simulink model "Gripper2"  (R2013b)
settings: Solver=ode45  StartTime=0.0  StopTime=6  RelTol=1e-3
undefined symbols (not defined in the file): base, driveshaft, grip, GripperForSimulink, link1, link2, link3, link4, Part8, pin1, pin15mm, pin50mm, RootGround, RootPart
libraries: mblibv1 x65, fl_lib x10, nesl_utility x5, elec_lib x1, simulink x1
(part 2 of 2)

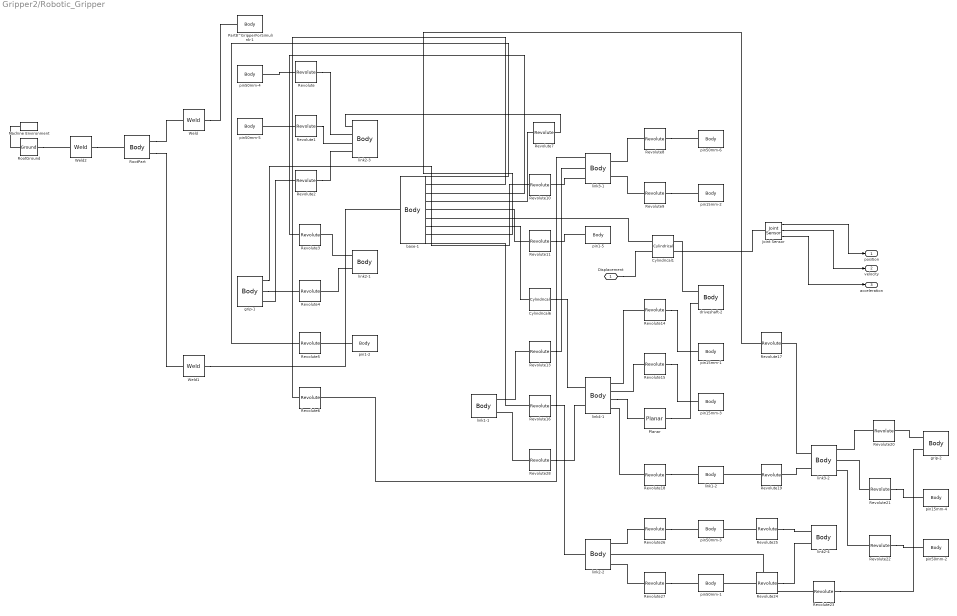
== system Gripper2/Robotic_Gripper ==
  Cylindrical1 : mblibv1/Joints/Cylindrical  LConnTagsString=__newl0|SA1  RConnTagsString=__newr0|SA1  UpdateFromCAD=on  NumSAPorts=2  CutJoint=off  MarkAsCut=off  Primitives=prismatic  PrimitiveProps=P1$World$[1 0 0]$prismatic#R1$World$[1 0 0]$revolute  DialogClass=JointBlock  P1Axis=[1 0 0]  R1Axis=[1 0 0]
  Cylindrical6 : mblibv1/Joints/Cylindrical  LConnTagsString=__newl0  RConnTagsString=__newr0  UpdateFromCAD=on  PMImportedID=base-1:-:link4-1  NumSAPorts=0  CutJoint=off  MarkAsCut=off  Primitives=prismatic  PrimitiveProps=P1$World$[1 0 0]$prismatic#R1$World$[1 0 0]$revolute  DialogClass=JointBlock  P1Axis=[1 0 0]  R1Axis=[1 0 0]
  Joint Sensor : mblibv1/Sensors &  Actuators/Joint Sensor  UpdateFromCAD=off  PhysicalDomain=Mechanical  PortType=blob  Muxed=off  Pose=off  Angle=on  AngleUnits=deg  ArcVelocity=off  ArcVelocityUnits=deg/s  ArcAcceleration=off  ArcAccelerationUnits=deg/s^2  CoordPosition=on  CoordPositionUnits=m  Velocity=on  VelocityUnits=m/s  Acceleration=on  AccelerationUnits=m/s^2  Quaternion=on  QuaternionDT=off  QuaternionDDT=off  QuaternionUnits=off  OutputVector=[1]  ActiveIO=on  Width=3  DialogClass=MechanicalSensorBlock  Primitive=P1  Force=off  ForceUnits=N  Torque=off  TorqueUnits=N*m  ReferenceFrame=Absolute (World)  ReactionSensedSide=Base  ReactionReferenceFrame=Absolute (World)  ReactionForce=off  ReactionForceUnits=N  ReactionMoment=off  ReactionMomentUnits=N*m
  Machine Environment : mblibv1/Bodies/Machine Environment  PortType=env  PhysicalDomain=Mechanical  DialogTemplateClass=MECH.MachineEnvironment  SyncWhenCopied=off  Gravity=[0 0 0]  GravityUnits=m/s^2  GravityAsSignal=off  Dimensionality=Auto-detect  AnalysisType=Forward dynamics  LinearAssemblyTolerance=1e-3  LinearAssemblyToleranceUnits=m  AngularAssemblyTolerance=1e-3  AngularAssemblyToleranceUnits=rad  ConstraintSolverType=Stabilizing  ConstraintRelTolerance=1e-4  ConstraintAbsTolerance=1e-4  UseRobustSingularityHandling=off  RedundancyAnalysisToleranceType=Automatically select tolerance  RedundancyAnalysisTolerance=1e-14  StatePerturbationType=Fixed  PerturbationSize=1e-5  VisualizeMachine=on  BodyVisualizationType=Use model default body geometries  BodyColorSelMode=Use model default  DefaultBodyColor=[1 0 0]
  Part8^GripperForSimulink-1 : mblibv1/Bodies/Body  LConnTagsString=CS2  UpdateFromCAD=on  PMImportedID=Part8^GripperForSimulink-1  DialogClass=MechanicalBodyBlock  Mass=0  MassUnits=kg  InertiaUnits=kg*m^2  Inertia=[0,0,0;0,0,0;0,0,0]  Shape=Cylinder  ShapeDims=[1 1]  ShapeUnits=m  ShapeUse=false  Density=1  DensityUnits=kg/m^3  DensityUse=false  GraphicsMode=GFXFILE  GraphicsFileName=GripperForSimulink - Part8^GripperForSimulink-1.STL  BodyColorSelMode=COLORPALETTE  BodyColor=[0.792157;0.819608;0.933333]  AttachedToCS=CS1  CG=Right$CG$[0 0 0]$WORLD$WORLD$m$[1 0 0;0 1 0;0 0 1]$3x3 Transform$rad$WORLD$false$Part8^GripperForSimulink-1::CG(AUTOGEN)  WorkingFrames=Right$CS1$[0 0 0]$WORLD$WORLD$m$[1 0 0;0 1 0;0 0 1]$3x3 Transform$rad$WORLD$false$Part8^GripperForSimulink-1::CS1(AUTOGEN)#Left$CS2$[0 0 0]$WORLD$WORLD$m$[1 0 0;0 1 0;0 0 1]$3x3 Transform$rad$WORLD$true$GripperForSimulink/RootPart:-:Part8^GripperForSimulink-1::Part8^GripperForSimulink-1(AUTOGEN)  CGPos=[0 0 0]  CGRot=[1 0 0;0 1 0;0 0 1]  CS0Pos=[]  CS0Rot=[]  CS1Pos=[0 0 0]  CS1Rot=[1 0 0;0 1 0;0 0 1]  CS2Pos=[0 0 0]  CS2Rot=[1 0 0;0 1 0;0 0 1]  CS3Pos=[]  CS3Rot=[]  CS4Pos=[]  CS4Rot=[]  CS5Pos=[]  CS5Rot=[]  CS6Pos=[]  CS6Rot=[]  CS7Pos=[]  CS7Rot=[]  CS8Pos=[]  CS8Rot=[]  CS9Pos=[]  CS9Rot=[]  CS10Pos=[]  CS10Rot=[]  CS11Pos=[]  CS11Rot=[]  CS12Pos=[]  CS12Rot=[]  CS13Pos=[]  CS13Rot=[]  CS14Pos=[]  CS14Rot=[]  CS15Pos=[]  CS15Rot=[]  CS16Pos=[]  CS16Rot=[]  CS17Pos=[]  CS17Rot=[]  CS18Pos=[]  CS18Rot=[]  CS19Pos=[]  CS19Rot=[]  CS20Pos=[]  CS20Rot=[]
  Planar : mblibv1/Joints/Planar  LConnTagsString=__newl0  RConnTagsString=__newr0  UpdateFromCAD=on  PMImportedID=driveshaft-2:-:link4-1  NumSAPorts=0  CutJoint=off  MarkAsCut=off  Primitives=prismatic_prismatic  PrimitiveProps=P1$World$[0,1,0]$prismatic#P2$World$[0,0,1]$prismatic#R1$World$[1,0,0]$revolute  DialogClass=JointBlock  P1Axis=[0,1,0]  P2Axis=[0,0,1]  R1Axis=[1,0,0]
  Revolute{,1..11,13..28} (28 alike) : mblibv1/Joints/Revolute  LConnTagsString=__newl0  RConnTagsString=__newr0  UpdateFromCAD=off  NumSAPorts=0  CutJoint=off  MarkAsCut=off  Primitives=prismatic  PrimitiveProps=R1$WORLD$[0 0 1]$revolute  DialogClass=JointBlock  R1Axis=[0 0 1]
  RootGround : mblibv1/Bodies/Ground  UpdateFromCAD=on  PMImportedID=RootGround  LeftPortType=env  RightPortType=workingframe  PhysicalDomain=Mechanical  DialogClass=GroundBlock  CoordPosition=[0.0300865,-0.00078351,0.0233471]  CoordPositionUnits=m  StateVectorMgrId=4  MachineId=[5 0]  ShowEnvPort=on  ParameterChecksum=[2079004459, 1115045925, 2663181990, 1030677230]  TopologyChecksum=[1966038930, 1606209126, 1995956594, 3418706587]
  RootPart : mblibv1/Bodies/Body  LConnTagsString=CS4  RConnTagsString=CS2|CS3  UpdateFromCAD=on  PMImportedID=GripperForSimulink/RootPart  DialogClass=MechanicalBodyBlock  Mass=0  MassUnits=kg  InertiaUnits=kg*m^2  Inertia=[0,0,0;0,0,0;0,0,0]  Shape=Cylinder  ShapeDims=[1 1]  ShapeUnits=m  ShapeUse=false  Density=1  DensityUnits=kg/m^3  DensityUse=false  GraphicsMode=MACHINE_DEFAULT  BodyColorSelMode=MACHINE_DEFAULT  BodyColor=[1;0;0]  AttachedToCS=CS1  CG=Right$CG$[0.0300865 -0.00078351 0.0233471]$WORLD$WORLD$m$[1 0 0;0 1 0;0 0 1]$3x3 Transform$rad$WORLD$false$GripperForSimulink/RootPart::CG(AUTOGEN)  WorkingFrames=Right$CS1$[0 0 0]$WORLD$WORLD$m$[1 0 0;0 1 0;0 0 1]$3x3 Transform$rad$WORLD$false$GripperForSimulink/RootPart::CS1(AUTOGEN)#Right$CS2$[0 0 0]$WORLD$WORLD$m$[1 0 0;0 1 0;0 0 1]$3x3 Transform$rad$WORLD$true$GripperForSimulink/RootPart:-:Part8^GripperForSimulink-1::GripperForSimulink/RootPart(AUTOGEN)#Right$CS3$[-0.043944 -0.000782836 0.0233426]$WORLD$WORLD$m$[1 0 0;0 1 0;0 0 1]$3x3 Transform$rad$WORLD$true$GripperForSimulink/RootPart:-:base-1::GripperForSimulink/RootPart(AUTOGEN)#Left$CS4$[0.0300865 -0.00078351 0.0233471]$WORLD$WORLD$m$[1 0 0;0 1 0;0 0 1]$3x3 Transform$rad$WORLD$true$GripperForSimulink/RootPart:-:RootGround::GripperForSimulink/RootPart(AUTOGEN)  CGPos=[0.0300865 -0.00078351 0.0233471]  CGRot=[1 0 0;0 1 0;0 0 1]  CS0Pos=[]  CS0Rot=[]  CS1Pos=[0 0 0]  CS1Rot=[1 0 0;0 1 0;0 0 1]  CS2Pos=[0 0 0]  CS2Rot=[1 0 0;0 1 0;0 0 1]  CS3Pos=[-0.043944 -0.000782836 0.0233426]  CS3Rot=[1 0 0;0 1 0;0 0 1]  CS4Pos=[0.0300865 -0.00078351 0.0233471]  CS4Rot=[1 0 0;0 1 0;0 0 1]  CS5Pos=[]  CS5Rot=[]  CS6Pos=[]  CS6Rot=[]  CS7Pos=[]  CS7Rot=[]  CS8Pos=[]  CS8Rot=[]  CS9Pos=[]  CS9Rot=[]  CS10Pos=[]  CS10Rot=[]  CS11Pos=[]  CS11Rot=[]  CS12Pos=[]  CS12Rot=[]  CS13Pos=[]  CS13Rot=[]  CS14Pos=[]  CS14Rot=[]  CS15Pos=[]  CS15Rot=[]  CS16Pos=[]  CS16Rot=[]  CS17Pos=[]  CS17Rot=[]  CS18Pos=[]  CS18Rot=[]  CS19Pos=[]  CS19Rot=[]  CS20Pos=[]  CS20Rot=[]
  Weld : mblibv1/Joints/Weld  LConnTagsString=__newl0  RConnTagsString=__newr0  UpdateFromCAD=on  PMImportedID=GripperForSimulink/RootPart:-:Part8^GripperForSimulink-1  NumSAPorts=0  CutJoint=off  MarkAsCut=off  Primitives=weld  PrimitiveProps=W$WORLD$[0.57735,0.57735,0.57735]$weld  DialogClass=JointBlock  WAxis=[0.57735,0.57735,0.57735]
  Weld1 : mblibv1/Joints/Weld  LConnTagsString=__newl0  RConnTagsString=__newr0  UpdateFromCAD=on  PMImportedID=GripperForSimulink/RootPart:-:base-1  NumSAPorts=0  CutJoint=off  MarkAsCut=off  Primitives=weld  PrimitiveProps=W$WORLD$[0.57735,0.57735,0.57735]$weld  DialogClass=JointBlock  WAxis=[0.57735,0.57735,0.57735]
  Weld2 : mblibv1/Joints/Weld  LConnTagsString=__newl0  RConnTagsString=__newr0  UpdateFromCAD=on  PMImportedID=GripperForSimulink/RootPart:-:RootGround  NumSAPorts=0  CutJoint=off  MarkAsCut=off  Primitives=weld  PrimitiveProps=W$WORLD$[0.57735,0.57735,0.57735]$weld  DialogClass=JointBlock  WAxis=[0.57735,0.57735,0.57735]
  base-1 : mblibv1/Bodies/Body  LConnTagsString=CS2  RConnTagsString=CS3|CS4|CS5|CS6|CS7|CS8|CS9|CS10|CS11  UpdateFromCAD=on  PMImportedID=base-1  DialogClass=MechanicalBodyBlock  Mass=0.147606  MassUnits=kg  InertiaUnits=kg*m^2  Inertia=[0.000194575,0,0;0,0.000219515,0;0,0,0.000354174]  Shape=Cylinder  ShapeDims=[1 1]  ShapeUnits=m  ShapeUse=false  Density=1  DensityUnits=kg/m^3  DensityUse=false  GraphicsMode=GFXFILE  GraphicsFileName=GripperForSimulink - base-1.STL  BodyColorSelMode=COLORPALETTE  BodyColor=[0.792157;0.819608;0.933333]  AttachedToCS=CS1  CG=Right$CG$[-0.043944 -0.000782836 0.0233426]$WORLD$WORLD$m$[1 0 0;0 1 0;0 0 1]$3x3 Transform$rad$WORLD$false$base-1::CG(AUTOGEN)  WorkingFrames=Right$CS1$[6.48367e-05 0.0413573 0.00359264]$WORLD$WORLD$m$[1 0 0;0 1 0;0 0 1]$3x3 Transform$rad$WORLD$false$base-1::CS1(AUTOGEN)#Left$CS2$[-0.043944 -0.000782836 0.0233426]$WORLD$WORLD$m$[1 0 0;0 1 0;0 0 1]$3x3 Transform$rad$WORLD$true$GripperForSimulink/RootPart:-:base-1::base-1(AUTOGEN)#Right$CS3$[-0.00973859 0.0614627 0.0108426]$WORLD$WORLD$m$[1 0 0;0 1 0;0 0 1]$3x3 Transform$rad$WORLD$true$base-1:-:pin1-2::base-1(AUTOGEN)#Right$CS4$[-0.00973859 0.0614627 0.0358426]$WORLD$WORLD$m$[1 0 0;0 1 0;0 0 1]$3x3 Transform$rad$WORLD$true$base-1:-:link3-1::base-1(AUTOGEN)#Right$CS5$[0.00656063 0.0362648 0.0358426]$WORLD$WORLD$m$[1 0 0;0 1 0;0 0 1]$3x3 Transform$rad$WORLD$true$base-1:-:link2-1::base-1(AUTOGEN)#Right$CS6$[0.00656063 0.0362648 0.0108426]$WORLD$WORLD$m$[1 0 0;0 1 0;0 0 1]$3x3 Transform$rad$WORLD$true$base-1:-:link2-3::base-1(AUTOGEN)#Right$CS7$[-0.00973859 -0.0630284 0.0358426]$WORLD$WORLD$m$[1 0 0;0 1 0;0 0 1]$3x3 Transform$rad$WORLD$true$base-1:-:pin1-5::base-1(AUTOGEN)#Right$CS8$[0.0165606 -0.000782836 0.0233426]$WORLD$WORLD$m$[1 0 0;0 1 0;0 0 1]$3x3 Transform$rad$WORLD$true$base-1:-:driveshaft-2::base-1(AUTOGEN)#Right$CS9$[0.0165606 -0.000782836 0.0233426]$WORLD$WORLD$m$[1 0 0;0 1 0;0 0 1]$3x3 Transform$rad$WORLD$true$base-1:-:link4-1::base-1(AUTOGEN)#Right$CS10$[-0.00973859 -0.0630284 0.0358426]$WORLD$WORLD$m$[1 0 0;0 1 0;0 0 1]$3x3 Transform$rad$WORLD$true$base-1:-:link3-2::base-1(AUTOGEN)#Right$CS11$[0.00656063 -0.0378305 0.0108426]$WORLD$WORLD$m$[1 0 0;0 1 0;0 0 1]$3x3 Transform$rad$WORLD$true$base-1:-:link2-2::base-1(AUTOGEN)  CGPos=[-0.043944 -0.000782836 0.0233426]  CGRot=[1 0 0;0 1 0;0 0 1]  CS0Pos=[]  CS0Rot=[]  CS1Pos=[6.48367e-05 0.0413573 0.00359264]  CS1Rot=[1 0 0;0 1 0;0 0 1]  CS2Pos=[-0.043944 -0.000782836 0.0233426]  CS2Rot=[1 0 0;0 1 0;0 0 1]  CS3Pos=[-0.00973859 0.0614627 0.0108426]  CS3Rot=[1 0 0;0 1 0;0 0 1]  CS4Pos=[-0.00973859 0.0614627 0.0358426]  CS4Rot=[1 0 0;0 1 0;0 0 1]  CS5Pos=[0.00656063 0.0362648 0.0358426]  CS5Rot=[1 0 0;0 1 0;0 0 1]  CS6Pos=[0.00656063 0.0362648 0.0108426]  CS6Rot=[1 0 0;0 1 0;0 0 1]  CS7Pos=[-0.00973859 -0.0630284 0.0358426]  CS7Rot=[1 0 0;0 1 0;0 0 1]  CS8Pos=[0.0165606 -0.000782836 0.0233426]  CS8Rot=[1 0 0;0 1 0;0 0 1]  CS9Pos=[0.0165606 -0.000782836 0.0233426]  CS9Rot=[1 0 0;0 1 0;0 0 1]  CS10Pos=[-0.00973859 -0.0630284 0.0358426]  CS10Rot=[1 0 0;0 1 0;0 0 1]  CS11Pos=[0.00656063 -0.0378305 0.0108426]  CS11Rot=[1 0 0;0 1 0;0 0 1]  CS12Pos=[]  CS12Rot=[]  CS13Pos=[]  CS13Rot=[]  CS14Pos=[]  CS14Rot=[]  CS15Pos=[]  CS15Rot=[]  CS16Pos=[]  CS16Rot=[]  CS17Pos=[]  CS17Rot=[]  CS18Pos=[]  CS18Rot=[]  CS19Pos=[]  CS19Rot=[]  CS20Pos=[]  CS20Rot=[]
  driveshaft-2 : mblibv1/Bodies/Body  LConnTagsString=CS2|CS3  RConnTagsString=CS5|CS4  UpdateFromCAD=on  PMImportedID=driveshaft-2  DialogClass=MechanicalBodyBlock  Mass=0.014633  MassUnits=kg  InertiaUnits=kg*m^2  Inertia=[2.0586e-05,0,2.10306e-08;0,2.05843e-05,0;2.10306e-08,0,2.62788e-07]  Shape=Cylinder  ShapeDims=[1 1]  ShapeUnits=m  ShapeUse=false  Density=1  DensityUnits=kg/m^3  DensityUse=false  GraphicsMode=GFXFILE  GraphicsFileName=GripperForSimulink - driveshaft-2.STL  BodyColorSelMode=COLORPALETTE  BodyColor=[0.79216 0.81961 0.93333]  AttachedToCS=CS1  CG=Right$CG$[-0.0900725 -0.000805943 0.0233368]$WORLD$WORLD$m$[0 0 -1;0.969279 0.245962 0;0.245962 -0.969279 0]$3x3 Transform$rad$WORLD$false$driveshaft-2::CG(AUTOGEN)  WorkingFrames=Right$CS5$[-0.0900725 -0.000805943 0.0233368]$WORLD$WORLD$m$[0 0 -1;0.969279 0.245962 0;0.245962 -0.969279 0]$3x3 Transform$rad$WORLD$true$none#Right$CS4$[-0.0900725 -0.000805943 0.0233368]$WORLD$WORLD$m$[0 0 -1;0.969279 0.245962 0;0.245962 -0.969279 0]$3x3 Transform$rad$WORLD$true$none#Right$CS1$[-0.0253581 -0.000782836 0.0233426]$WORLD$WORLD$m$[0 0 -1;0.969279 0.245962 0;0.245962 -0.969279 0]$3x3 Transform$rad$WORLD$false$driveshaft-2::CS1(AUTOGEN)#Left$CS2$[0.0165606 -0.000782836 0.0233426]$WORLD$WORLD$m$[1 0 0;0 1 0;0 0 1]$3x3 Transform$rad$WORLD$true$base-1:-:driveshaft-2::driveshaft-2(AUTOGEN)#Left$CS3$[-0.0253581 -0.0132828 0.0358426]$WORLD$WORLD$m$[1 0 0;0 1 0;0 0 1]$3x3 Transform$rad$WORLD$true$driveshaft-2:-:link4-1::driveshaft-2(AUTOGEN)  CGPos=[-0.0900725 -0.000805943 0.0233368]  CGRot=[0 0 -1;0.969279 0.245962 0;0.245962 -0.969279 0]  CS0Pos=[]  CS0Rot=[]  CS1Pos=[-0.0253581 -0.000782836 0.0233426]  CS1Rot=[0 0 -1;0.969279 0.245962 0;0.245962 -0.969279 0]  CS2Pos=[0.0165606 -0.000782836 0.0233426]  CS2Rot=[1 0 0;0 1 0;0 0 1]  CS3Pos=[-0.0253581 -0.0132828 0.0358426]  CS3Rot=[1 0 0;0 1 0;0 0 1]  CS4Pos=[-0.0900725 -0.000805943 0.0233368]  CS4Rot=[0 0 -1;0.969279 0.245962 0;0.245962 -0.969279 0]  CS5Pos=[-0.0900725 -0.000805943 0.0233368]  CS5Rot=[0 0 -1;0.969279 0.245962 0;0.245962 -0.969279 0]  CS6Pos=[]  CS6Rot=[]  CS7Pos=[]  CS7Rot=[]  CS8Pos=[]  CS8Rot=[]  CS9Pos=[]  CS9Rot=[]  CS10Pos=[]  CS10Rot=[]  CS11Pos=[]  CS11Rot=[]  CS12Pos=[]  CS12Rot=[]  CS13Pos=[]  CS13Rot=[]  CS14Pos=[]  CS14Rot=[]  CS15Pos=[]  CS15Rot=[]  CS16Pos=[]  CS16Rot=[]  CS17Pos=[]  CS17Rot=[]  CS18Pos=[]  CS18Rot=[]  CS19Pos=[]  CS19Rot=[]  CS20Pos=[]  CS20Rot=[]
  grip-1 : mblibv1/Bodies/Body  RConnTagsString=CS2|CS3|CS4  UpdateFromCAD=on  PMImportedID=grip-1  DialogClass=MechanicalBodyBlock  Mass=0.126042  MassUnits=kg  InertiaUnits=kg*m^2  Inertia=[3.20073e-05,1.79918e-05,0;1.79918e-05,0.000117875,0;0,0,0.000116271]  Shape=Cylinder  ShapeDims=[1 1]  ShapeUnits=m  ShapeUse=false  Density=1  DensityUnits=kg/m^3  DensityUse=false  GraphicsMode=GFXFILE  GraphicsFileName=GripperForSimulink - grip-1.STL  BodyColorSelMode=COLORPALETTE  BodyColor=[0.792157;0.819608;0.933333]  AttachedToCS=CS1  CG=Right$CG$[0.0889703 0.0472336 0.0233426]$WORLD$WORLD$m$[0.99978 0.0209596 0;-0.0209596 0.99978 0;0 0 1]$3x3 Transform$rad$WORLD$false$grip-1::CG(AUTOGEN)  WorkingFrames=Right$CS1$[0.0895492 0.047536 0.00334264]$WORLD$WORLD$m$[0.99978 0.0209596 0;-0.0209596 0.99978 0;0 0 1]$3x3 Transform$rad$WORLD$false$grip-1::CS1(AUTOGEN)#Right$CS2$[0.0480334 0.0678885 0.0433426]$WORLD$WORLD$m$[1 0 0;0 1 0;0 0 1]$3x3 Transform$rad$WORLD$true$grip-1:-:link3-1::grip-1(AUTOGEN)#Right$CS3$[0.0560713 0.043243 0.0433426]$WORLD$WORLD$m$[1 0 0;0 1 0;0 0 1]$3x3 Transform$rad$WORLD$true$grip-1:-:link2-1::grip-1(AUTOGEN)#Right$CS4$[0.0560713 0.043243 0.0433426]$WORLD$WORLD$m$[1 0 0;0 1 0;0 0 1]$3x3 Transform$rad$WORLD$true$grip-1:-:link2-3::grip-1(AUTOGEN)  CGPos=[0.0889703 0.0472336 0.0233426]  CGRot=[0.99978 0.0209596 0;-0.0209596 0.99978 0;0 0 1]  CS0Pos=[]  CS0Rot=[]  CS1Pos=[0.0895492 0.047536 0.00334264]  CS1Rot=[0.99978 0.0209596 0;-0.0209596 0.99978 0;0 0 1]  CS2Pos=[0.0480334 0.0678885 0.0433426]  CS2Rot=[1 0 0;0 1 0;0 0 1]  CS3Pos=[0.0560713 0.043243 0.0433426]  CS3Rot=[1 0 0;0 1 0;0 0 1]  CS4Pos=[0.0560713 0.043243 0.0433426]  CS4Rot=[1 0 0;0 1 0;0 0 1]  CS5Pos=[]  CS5Rot=[]  CS6Pos=[]  CS6Rot=[]  CS7Pos=[]  CS7Rot=[]  CS8Pos=[]  CS8Rot=[]  CS9Pos=[]  CS9Rot=[]  CS10Pos=[]  CS10Rot=[]  CS11Pos=[]  CS11Rot=[]  CS12Pos=[]  CS12Rot=[]  CS13Pos=[]  CS13Rot=[]  CS14Pos=[]  CS14Rot=[]  CS15Pos=[]  CS15Rot=[]  CS16Pos=[]  CS16Rot=[]  CS17Pos=[]  CS17Rot=[]  CS18Pos=[]  CS18Rot=[]  CS19Pos=[]  CS19Rot=[]  CS20Pos=[]  CS20Rot=[]
  grip-2 : mblibv1/Bodies/Body  LConnTagsString=CS2|CS3  UpdateFromCAD=on  PMImportedID=grip-2  DialogClass=MechanicalBodyBlock  Mass=0.126042  MassUnits=kg  InertiaUnits=kg*m^2  Inertia=[3.20073e-05,1.79918e-05,0;1.79918e-05,0.000117875,0;0,0,0.000116271]  Shape=Cylinder  ShapeDims=[1 1]  ShapeUnits=m  ShapeUse=false  Density=1  DensityUnits=kg/m^3  DensityUse=false  GraphicsMode=GFXFILE  GraphicsFileName=GripperForSimulink - grip-2.STL  BodyColorSelMode=COLORPALETTE  BodyColor=[0.792157;0.819608;0.933333]  AttachedToCS=CS1  CG=Right$CG$[0.0889703 -0.0487992 0.0233426]$WORLD$WORLD$m$[0.99978 0.0209596 0;0.0209596 -0.99978 0;0 0 -1]$3x3 Transform$rad$WORLD$false$grip-2::CG(AUTOGEN)  WorkingFrames=Right$CS1$[0.0895492 -0.0491017 0.0433426]$WORLD$WORLD$m$[0.99978 0.0209596 0;0.0209596 -0.99978 0;0 0 -1]$3x3 Transform$rad$WORLD$false$grip-2::CS1(AUTOGEN)#Left$CS2$[0.0480334 -0.0694542 0.0483426]$WORLD$WORLD$m$[1 0 0;0 1 0;0 0 1]$3x3 Transform$rad$WORLD$true$grip-2:-:link3-2::grip-2(AUTOGEN)#Left$CS3$[0.0560713 -0.0448086 0.0433426]$WORLD$WORLD$m$[1 0 0;0 1 0;0 0 1]$3x3 Transform$rad$WORLD$true$grip-2:-:link2-2::grip-2(AUTOGEN)  CGPos=[0.0889703 -0.0487992 0.0233426]  CGRot=[0.99978 0.0209596 0;0.0209596 -0.99978 0;0 0 -1]  CS0Pos=[]  CS0Rot=[]  CS1Pos=[0.0895492 -0.0491017 0.0433426]  CS1Rot=[0.99978 0.0209596 0;0.0209596 -0.99978 0;0 0 -1]  CS2Pos=[0.0480334 -0.0694542 0.0483426]  CS2Rot=[1 0 0;0 1 0;0 0 1]  CS3Pos=[0.0560713 -0.0448086 0.0433426]  CS3Rot=[1 0 0;0 1 0;0 0 1]  CS4Pos=[]  CS4Rot=[]  CS5Pos=[]  CS5Rot=[]  CS6Pos=[]  CS6Rot=[]  CS7Pos=[]  CS7Rot=[]  CS8Pos=[]  CS8Rot=[]  CS9Pos=[]  CS9Rot=[]  CS10Pos=[]  CS10Rot=[]  CS11Pos=[]  CS11Rot=[]  CS12Pos=[]  CS12Rot=[]  CS13Pos=[]  CS13Rot=[]  CS14Pos=[]  CS14Rot=[]  CS15Pos=[]  CS15Rot=[]  CS16Pos=[]  CS16Rot=[]  CS17Pos=[]  CS17Rot=[]  CS18Pos=[]  CS18Rot=[]  CS19Pos=[]  CS19Rot=[]  CS20Pos=[]  CS20Rot=[]
  link1-1 : mblibv1/Bodies/Body  RConnTagsString=CS2|CS3  UpdateFromCAD=on  PMImportedID=link1-1  DialogClass=MechanicalBodyBlock  Mass=0.00188092  MassUnits=kg  InertiaUnits=kg*m^2  Inertia=[4.24582e-08,0,0;0,1.58675e-07,0;0,0,1.93296e-07]  Shape=Cylinder  ShapeDims=[1 1]  ShapeUnits=m  ShapeUse=false  Density=1  DensityUnits=kg/m^3  DensityUse=false  GraphicsMode=GFXFILE  GraphicsFileName=GripperForSimulink - link1-1.STL  BodyColorSelMode=COLORPALETTE  BodyColor=[0.752941;0.752941;0.752941]  AttachedToCS=CS1  CG=Right$CG$[-0.0278863 0.0284656 0.0233426]$WORLD$WORLD$m$[0.997172 -0.0751545 0;-0.0751545 -0.997172 0;0 0 -1]$3x3 Transform$rad$WORLD$false$link1-1::CG(AUTOGEN)  WorkingFrames=Right$CS1$[-0.0384217 0.0217384 0.0258426]$WORLD$WORLD$m$[0.997172 -0.0751545 0;-0.0751545 -0.997172 0;0 0 -1]$3x3 Transform$rad$WORLD$false$link1-1::CS1(AUTOGEN)#Right$CS2$[-0.0179146 0.0277141 0.0208426]$WORLD$WORLD$m$[1 0 0;0 1 0;0 0 1]$3x3 Transform$rad$WORLD$true$link1-1:-:link3-1::link1-1(AUTOGEN)#Right$CS3$[-0.0378581 0.0292172 0.0208426]$WORLD$WORLD$m$[1 0 0;0 1 0;0 0 1]$3x3 Transform$rad$WORLD$true$link1-1:-:link4-1::link1-1(AUTOGEN)  CGPos=[-0.0278863 0.0284656 0.0233426]  CGRot=[0.997172 -0.0751545 0;-0.0751545 -0.997172 0;0 0 -1]  CS0Pos=[]  CS0Rot=[]  CS1Pos=[-0.0384217 0.0217384 0.0258426]  CS1Rot=[0.997172 -0.0751545 0;-0.0751545 -0.997172 0;0 0 -1]  CS2Pos=[-0.0179146 0.0277141 0.0208426]  CS2Rot=[1 0 0;0 1 0;0 0 1]  CS3Pos=[-0.0378581 0.0292172 0.0208426]  CS3Rot=[1 0 0;0 1 0;0 0 1]  CS4Pos=[]  CS4Rot=[]  CS5Pos=[]  CS5Rot=[]  CS6Pos=[]  CS6Rot=[]  CS7Pos=[]  CS7Rot=[]  CS8Pos=[]  CS8Rot=[]  CS9Pos=[]  CS9Rot=[]  CS10Pos=[]  CS10Rot=[]  CS11Pos=[]  CS11Rot=[]  CS12Pos=[]  CS12Rot=[]  CS13Pos=[]  CS13Rot=[]  CS14Pos=[]  CS14Rot=[]  CS15Pos=[]  CS15Rot=[]  CS16Pos=[]  CS16Rot=[]  CS17Pos=[]  CS17Rot=[]  CS18Pos=[]  CS18Rot=[]  CS19Pos=[]  CS19Rot=[]  CS20Pos=[]  CS20Rot=[]
  link1-2 : mblibv1/Bodies/Body  LConnTagsString=CS2  RConnTagsString=CS3  UpdateFromCAD=on  PMImportedID=link1-2  DialogClass=MechanicalBodyBlock  Mass=0.00188092  MassUnits=kg  InertiaUnits=kg*m^2  Inertia=[4.24582e-08,0,0;0,1.58675e-07,0;0,0,1.93296e-07]  Shape=Cylinder  ShapeDims=[1 1]  ShapeUnits=m  ShapeUse=false  Density=1  DensityUnits=kg/m^3  DensityUse=false  GraphicsMode=GFXFILE  GraphicsFileName=GripperForSimulink - link1-2.STL  BodyColorSelMode=COLORPALETTE  BodyColor=[0.752941;0.752941;0.752941]  AttachedToCS=CS1  CG=Right$CG$[-0.0278863 -0.0300313 0.0233426]$WORLD$WORLD$m$[0.997172 0.0751545 0;0.0751545 -0.997172 0;0 0 -1]$3x3 Transform$rad$WORLD$false$link1-2::CG(AUTOGEN)  WorkingFrames=Right$CS1$[-0.0372944 -0.0382616 0.0258426]$WORLD$WORLD$m$[0.997172 0.0751545 0;0.0751545 -0.997172 0;0 0 -1]$3x3 Transform$rad$WORLD$false$link1-2::CS1(AUTOGEN)#Left$CS2$[-0.0378581 -0.0307828 0.0108426]$WORLD$WORLD$m$[1 0 0;0 1 0;0 0 1]$3x3 Transform$rad$WORLD$true$link1-2:-:link4-1::link1-2(AUTOGEN)#Right$CS3$[-0.0179146 -0.0292797 0.0208426]$WORLD$WORLD$m$[1 0 0;0 1 0;0 0 1]$3x3 Transform$rad$WORLD$true$link1-2:-:link3-2::link1-2(AUTOGEN)  CGPos=[-0.0278863 -0.0300313 0.0233426]  CGRot=[0.997172 0.0751545 0;0.0751545 -0.997172 0;0 0 -1]  CS0Pos=[]  CS0Rot=[]  CS1Pos=[-0.0372944 -0.0382616 0.0258426]  CS1Rot=[0.997172 0.0751545 0;0.0751545 -0.997172 0;0 0 -1]  CS2Pos=[-0.0378581 -0.0307828 0.0108426]  CS2Rot=[1 0 0;0 1 0;0 0 1]  CS3Pos=[-0.0179146 -0.0292797 0.0208426]  CS3Rot=[1 0 0;0 1 0;0 0 1]  CS4Pos=[]  CS4Rot=[]  CS5Pos=[]  CS5Rot=[]  CS6Pos=[]  CS6Rot=[]  CS7Pos=[]  CS7Rot=[]  CS8Pos=[]  CS8Rot=[]  CS9Pos=[]  CS9Rot=[]  CS10Pos=[]  CS10Rot=[]  CS11Pos=[]  CS11Rot=[]  CS12Pos=[]  CS12Rot=[]  CS13Pos=[]  CS13Rot=[]  CS14Pos=[]  CS14Rot=[]  CS15Pos=[]  CS15Rot=[]  CS16Pos=[]  CS16Rot=[]  CS17Pos=[]  CS17Rot=[]  CS18Pos=[]  CS18Rot=[]  CS19Pos=[]  CS19Rot=[]  CS20Pos=[]  CS20Rot=[]
  link2-1 : mblibv1/Bodies/Body  LConnTagsString=CS2|CS3  UpdateFromCAD=on  PMImportedID=link2-1  DialogClass=MechanicalBodyBlock  Mass=0.00413092  MassUnits=kg  InertiaUnits=kg*m^2  Inertia=[1.17897e-06,0,0;0,8.93332e-08,0;0,0,1.25109e-06]  Shape=Cylinder  ShapeDims=[1 1]  ShapeUnits=m  ShapeUse=false  Density=1  DensityUnits=kg/m^3  DensityUse=false  GraphicsMode=GFXFILE  GraphicsFileName=GripperForSimulink - link2-1.STL  BodyColorSelMode=COLORPALETTE  BodyColor=[0.792157;0.819608;0.933333]  AttachedToCS=CS1  CG=Right$CG$[0.031316 0.0397539 0.0458426]$WORLD$WORLD$m$[0.139562 0.990213 0;-0.990213 0.139562 0;0 0 1]$3x3 Transform$rad$WORLD$false$link2-1::CG(AUTOGEN)  WorkingFrames=Right$CS1$[0.0560713 0.043243 0.0433426]$WORLD$WORLD$m$[0.139562 0.990213 0;-0.990213 0.139562 0;0 0 1]$3x3 Transform$rad$WORLD$false$link2-1::CS1(AUTOGEN)#Left$CS2$[0.00656063 0.0362648 0.0358426]$WORLD$WORLD$m$[1 0 0;0 1 0;0 0 1]$3x3 Transform$rad$WORLD$true$base-1:-:link2-1::link2-1(AUTOGEN)#Left$CS3$[0.0560713 0.043243 0.0433426]$WORLD$WORLD$m$[1 0 0;0 1 0;0 0 1]$3x3 Transform$rad$WORLD$true$grip-1:-:link2-1::link2-1(AUTOGEN)  CGPos=[0.031316 0.0397539 0.0458426]  CGRot=[0.139562 0.990213 0;-0.990213 0.139562 0;0 0 1]  CS0Pos=[]  CS0Rot=[]  CS1Pos=[0.0560713 0.043243 0.0433426]  CS1Rot=[0.139562 0.990213 0;-0.990213 0.139562 0;0 0 1]  CS2Pos=[0.00656063 0.0362648 0.0358426]  CS2Rot=[1 0 0;0 1 0;0 0 1]  CS3Pos=[0.0560713 0.043243 0.0433426]  CS3Rot=[1 0 0;0 1 0;0 0 1]  CS4Pos=[]  CS4Rot=[]  CS5Pos=[]  CS5Rot=[]  CS6Pos=[]  CS6Rot=[]  CS7Pos=[]  CS7Rot=[]  CS8Pos=[]  CS8Rot=[]  CS9Pos=[]  CS9Rot=[]  CS10Pos=[]  CS10Rot=[]  CS11Pos=[]  CS11Rot=[]  CS12Pos=[]  CS12Rot=[]  CS13Pos=[]  CS13Rot=[]  CS14Pos=[]  CS14Rot=[]  CS15Pos=[]  CS15Rot=[]  CS16Pos=[]  CS16Rot=[]  CS17Pos=[]  CS17Rot=[]  CS18Pos=[]  CS18Rot=[]  CS19Pos=[]  CS19Rot=[]  CS20Pos=[]  CS20Rot=[]
  link2-2 : mblibv1/Bodies/Body  LConnTagsString=CS2  RConnTagsString=CS3|CS4|CS5  UpdateFromCAD=on  PMImportedID=link2-2  DialogClass=MechanicalBodyBlock  Mass=0.00413092  MassUnits=kg  InertiaUnits=kg*m^2  Inertia=[1.17897e-06,0,0;0,8.93332e-08,0;0,0,1.25109e-06]  Shape=Cylinder  ShapeDims=[1 1]  ShapeUnits=m  ShapeUse=false  Density=1  DensityUnits=kg/m^3  DensityUse=false  GraphicsMode=GFXFILE  GraphicsFileName=GripperForSimulink - link2-2.STL  BodyColorSelMode=COLORPALETTE  BodyColor=[0.792157;0.819608;0.933333]  AttachedToCS=CS1  CG=Right$CG$[0.031316 -0.0413196 0.0458426]$WORLD$WORLD$m$[-0.139562 -0.990213 0;-0.990213 0.139562 0;0 0 -1]$3x3 Transform$rad$WORLD$false$link2-2::CG(AUTOGEN)  WorkingFrames=Right$CS1$[0.00656063 -0.0378305 0.0483426]$WORLD$WORLD$m$[-0.139562 -0.990213 0;-0.990213 0.139562 0;0 0 -1]$3x3 Transform$rad$WORLD$false$link2-2::CS1(AUTOGEN)#Left$CS2$[0.00656063 -0.0378305 0.0108426]$WORLD$WORLD$m$[1 0 0;0 1 0;0 0 1]$3x3 Transform$rad$WORLD$true$base-1:-:link2-2::link2-2(AUTOGEN)#Right$CS3$[0.0560713 -0.0448086 0.0433426]$WORLD$WORLD$m$[1 0 0;0 1 0;0 0 1]$3x3 Transform$rad$WORLD$true$link2-2:-:pin50mm-3::link2-2(AUTOGEN)#Right$CS4$[0.0560713 -0.0448086 0.0433426]$WORLD$WORLD$m$[1 0 0;0 1 0;0 0 1]$3x3 Transform$rad$WORLD$true$grip-2:-:link2-2::link2-2(AUTOGEN)#Right$CS5$[0.00656063 -0.0378305 0.0433426]$WORLD$WORLD$m$[1 0 0;0 1 0;0 0 1]$3x3 Transform$rad$WORLD$true$link2-2:-:pin50mm-1::link2-2(AUTOGEN)  CGPos=[0.031316 -0.0413196 0.0458426]  CGRot=[-0.139562 -0.990213 0;-0.990213 0.139562 0;0 0 -1]  CS0Pos=[]  CS0Rot=[]  CS1Pos=[0.00656063 -0.0378305 0.0483426]  CS1Rot=[-0.139562 -0.990213 0;-0.990213 0.139562 0;0 0 -1]  CS2Pos=[0.00656063 -0.0378305 0.0108426]  CS2Rot=[1 0 0;0 1 0;0 0 1]  CS3Pos=[0.0560713 -0.0448086 0.0433426]  CS3Rot=[1 0 0;0 1 0;0 0 1]  CS4Pos=[0.0560713 -0.0448086 0.0433426]  CS4Rot=[1 0 0;0 1 0;0 0 1]  CS5Pos=[0.00656063 -0.0378305 0.0433426]  CS5Rot=[1 0 0;0 1 0;0 0 1]  CS6Pos=[]  CS6Rot=[]  CS7Pos=[]  CS7Rot=[]  CS8Pos=[]  CS8Rot=[]  CS9Pos=[]  CS9Rot=[]  CS10Pos=[]  CS10Rot=[]  CS11Pos=[]  CS11Rot=[]  CS12Pos=[]  CS12Rot=[]  CS13Pos=[]  CS13Rot=[]  CS14Pos=[]  CS14Rot=[]  CS15Pos=[]  CS15Rot=[]  CS16Pos=[]  CS16Rot=[]  CS17Pos=[]  CS17Rot=[]  CS18Pos=[]  CS18Rot=[]  CS19Pos=[]  CS19Rot=[]  CS20Pos=[]  CS20Rot=[]
  link2-3 : mblibv1/Bodies/Body  LConnTagsString=CS2|CS3|CS4|CS5  UpdateFromCAD=on  PMImportedID=link2-3  DialogClass=MechanicalBodyBlock  Mass=0.00413092  MassUnits=kg  InertiaUnits=kg*m^2  Inertia=[1.17897e-06,0,0;0,8.93332e-08,0;0,0,1.25109e-06]  Shape=Cylinder  ShapeDims=[1 1]  ShapeUnits=m  ShapeUse=false  Density=1  DensityUnits=kg/m^3  DensityUse=false  GraphicsMode=GFXFILE  GraphicsFileName=GripperForSimulink - link2-3.STL  BodyColorSelMode=COLORPALETTE  BodyColor=[0.792157;0.819608;0.933333]  AttachedToCS=CS1  CG=Right$CG$[0.031316 0.0397539 0.00109264]$WORLD$WORLD$m$[0.139562 -0.990213 0;-0.990213 -0.139562 0;0 0 -1]$3x3 Transform$rad$WORLD$false$link2-3::CG(AUTOGEN)  WorkingFrames=Right$CS1$[0.00656063 0.0362648 0.00359264]$WORLD$WORLD$m$[0.139562 -0.990213 0;-0.990213 -0.139562 0;0 0 -1]$3x3 Transform$rad$WORLD$false$link2-3::CS1(AUTOGEN)#Left$CS2$[0.00656063 0.0362648 0.0108426]$WORLD$WORLD$m$[1 0 0;0 1 0;0 0 1]$3x3 Transform$rad$WORLD$true$base-1:-:link2-3::link2-3(AUTOGEN)#Left$CS3$[0.00656063 0.0362648 0.0485926]$WORLD$WORLD$m$[1 0 0;0 1 0;0 0 1]$3x3 Transform$rad$WORLD$true$link2-3:-:pin50mm-4::link2-3(AUTOGEN)#Left$CS4$[0.0560713 0.043243 0.0485926]$WORLD$WORLD$m$[1 0 0;0 1 0;0 0 1]$3x3 Transform$rad$WORLD$true$link2-3:-:pin50mm-5::link2-3(AUTOGEN)#Left$CS5$[0.0560713 0.043243 0.0433426]$WORLD$WORLD$m$[1 0 0;0 1 0;0 0 1]$3x3 Transform$rad$WORLD$true$grip-1:-:link2-3::link2-3(AUTOGEN)  CGPos=[0.031316 0.0397539 0.00109264]  CGRot=[0.139562 -0.990213 0;-0.990213 -0.139562 0;0 0 -1]  CS0Pos=[]  CS0Rot=[]  CS1Pos=[0.00656063 0.0362648 0.00359264]  CS1Rot=[0.139562 -0.990213 0;-0.990213 -0.139562 0;0 0 -1]  CS2Pos=[0.00656063 0.0362648 0.0108426]  CS2Rot=[1 0 0;0 1 0;0 0 1]  CS3Pos=[0.00656063 0.0362648 0.0485926]  CS3Rot=[1 0 0;0 1 0;0 0 1]  CS4Pos=[0.0560713 0.043243 0.0485926]  CS4Rot=[1 0 0;0 1 0;0 0 1]  CS5Pos=[0.0560713 0.043243 0.0433426]  CS5Rot=[1 0 0;0 1 0;0 0 1]  CS6Pos=[]  CS6Rot=[]  CS7Pos=[]  CS7Rot=[]  CS8Pos=[]  CS8Rot=[]  CS9Pos=[]  CS9Rot=[]  CS10Pos=[]  CS10Rot=[]  CS11Pos=[]  CS11Rot=[]  CS12Pos=[]  CS12Rot=[]  CS13Pos=[]  CS13Rot=[]  CS14Pos=[]  CS14Rot=[]  CS15Pos=[]  CS15Rot=[]  CS16Pos=[]  CS16Rot=[]  CS17Pos=[]  CS17Rot=[]  CS18Pos=[]  CS18Rot=[]  CS19Pos=[]  CS19Rot=[]  CS20Pos=[]  CS20Rot=[]
  link2-4 : mblibv1/Bodies/Body  LConnTagsString=CS2|CS3  UpdateFromCAD=on  PMImportedID=link2-4  DialogClass=MechanicalBodyBlock  Mass=0.00413092  MassUnits=kg  InertiaUnits=kg*m^2  Inertia=[1.17897e-06,0,0;0,8.93332e-08,0;0,0,1.25109e-06]  Shape=Cylinder  ShapeDims=[1 1]  ShapeUnits=m  ShapeUse=false  Density=1  DensityUnits=kg/m^3  DensityUse=false  GraphicsMode=GFXFILE  GraphicsFileName=GripperForSimulink - link2-4.STL  BodyColorSelMode=COLORPALETTE  BodyColor=[0.792157;0.819608;0.933333]  AttachedToCS=CS1  CG=Right$CG$[0.031316 -0.0413196 0.00109264]$WORLD$WORLD$m$[0.139562 -0.990213 0;0.990213 0.139562 0;0 0 1]$3x3 Transform$rad$WORLD$false$link2-4::CG(AUTOGEN)  WorkingFrames=Right$CS1$[0.00656063 -0.0378305 -0.00140736]$WORLD$WORLD$m$[0.139562 -0.990213 0;0.990213 0.139562 0;0 0 1]$3x3 Transform$rad$WORLD$false$link2-4::CS1(AUTOGEN)#Left$CS2$[0.0560713 -0.0448086 0.0483426]$WORLD$WORLD$m$[1 0 0;0 1 0;0 0 1]$3x3 Transform$rad$WORLD$true$link2-4:-:pin50mm-3::link2-4(AUTOGEN)#Left$CS3$[0.00656063 -0.0378305 0.0483426]$WORLD$WORLD$m$[1 0 0;0 1 0;0 0 1]$3x3 Transform$rad$WORLD$true$link2-4:-:pin50mm-1::link2-4(AUTOGEN)  CGPos=[0.031316 -0.0413196 0.00109264]  CGRot=[0.139562 -0.990213 0;0.990213 0.139562 0;0 0 1]  CS0Pos=[]  CS0Rot=[]  CS1Pos=[0.00656063 -0.0378305 -0.00140736]  CS1Rot=[0.139562 -0.990213 0;0.990213 0.139562 0;0 0 1]  CS2Pos=[0.0560713 -0.0448086 0.0483426]  CS2Rot=[1 0 0;0 1 0;0 0 1]  CS3Pos=[0.00656063 -0.0378305 0.0483426]  CS3Rot=[1 0 0;0 1 0;0 0 1]  CS4Pos=[]  CS4Rot=[]  CS5Pos=[]  CS5Rot=[]  CS6Pos=[]  CS6Rot=[]  CS7Pos=[]  CS7Rot=[]  CS8Pos=[]  CS8Rot=[]  CS9Pos=[]  CS9Rot=[]  CS10Pos=[]  CS10Rot=[]  CS11Pos=[]  CS11Rot=[]  CS12Pos=[]  CS12Rot=[]  CS13Pos=[]  CS13Rot=[]  CS14Pos=[]  CS14Rot=[]  CS15Pos=[]  CS15Rot=[]  CS16Pos=[]  CS16Rot=[]  CS17Pos=[]  CS17Rot=[]  CS18Pos=[]  CS18Rot=[]  CS19Pos=[]  CS19Rot=[]  CS20Pos=[]  CS20Rot=[]
  link3-1 : mblibv1/Bodies/Body  LConnTagsString=CS2|CS4|CS6  RConnTagsString=CS3|CS5  UpdateFromCAD=on  PMImportedID=link3-1  DialogClass=MechanicalBodyBlock  Mass=0.0131167  MassUnits=kg  InertiaUnits=kg*m^2  Inertia=[7.39603e-06,-4.27092e-06,-1.73808e-08;-4.27092e-06,6.72647e-06,-1.85249e-08;-1.73808e-08,-1.85249e-08,1.01055e-05]  Shape=Cylinder  ShapeDims=[1 1]  ShapeUnits=m  ShapeUse=false  Density=1  DensityUnits=kg/m^3  DensityUse=false  GraphicsMode=GFXFILE  GraphicsFileName=GripperForSimulink - link3-1.STL  BodyColorSelMode=COLORPALETTE  BodyColor=[0.792157;0.819608;0.933333]  AttachedToCS=CS1  CG=Right$CG$[0.0128329 0.0566929 0.0234399]$WORLD$WORLD$m$[0.944391 0.328825 0;-0.328825 0.944391 0;0 0 1]$3x3 Transform$rad$WORLD$false$link3-1::CG(AUTOGEN)  WorkingFrames=Right$CS1$[-0.0214827 0.028881 0.0208426]$WORLD$WORLD$m$[0.944391 0.328825 0;-0.328825 0.944391 0;0 0 1]$3x3 Transform$rad$WORLD$false$link3-1::CS1(AUTOGEN)#Left$CS2$[-0.00973859 0.0614627 0.0358426]$WORLD$WORLD$m$[1 0 0;0 1 0;0 0 1]$3x3 Transform$rad$WORLD$true$base-1:-:link3-1::link3-1(AUTOGEN)#Right$CS3$[0.0480334 0.0678885 -0.00165736]$WORLD$WORLD$m$[1 0 0;0 1 0;0 0 1]$3x3 Transform$rad$WORLD$true$link3-1:-:pin50mm-6::link3-1(AUTOGEN)#Left$CS4$[-0.0179146 0.0277141 0.0208426]$WORLD$WORLD$m$[1 0 0;0 1 0;0 0 1]$3x3 Transform$rad$WORLD$true$link1-1:-:link3-1::link3-1(AUTOGEN)#Right$CS5$[-0.0179146 0.0277141 0.0258426]$WORLD$WORLD$m$[1 0 0;0 1 0;0 0 1]$3x3 Transform$rad$WORLD$true$link3-1:-:pin15mm-2::link3-1(AUTOGEN)#Left$CS6$[0.0480334 0.0678885 0.0433426]$WORLD$WORLD$m$[1 0 0;0 1 0;0 0 1]$3x3 Transform$rad$WORLD$true$grip-1:-:link3-1::link3-1(AUTOGEN)  CGPos=[0.0128329 0.0566929 0.0234399]  CGRot=[0.944391 0.328825 0;-0.328825 0.944391 0;0 0 1]  CS0Pos=[]  CS0Rot=[]  CS1Pos=[-0.0214827 0.028881 0.0208426]  CS1Rot=[0.944391 0.328825 0;-0.328825 0.944391 0;0 0 1]  CS2Pos=[-0.00973859 0.0614627 0.0358426]  CS2Rot=[1 0 0;0 1 0;0 0 1]  CS3Pos=[0.0480334 0.0678885 -0.00165736]  CS3Rot=[1 0 0;0 1 0;0 0 1]  CS4Pos=[-0.0179146 0.0277141 0.0208426]  CS4Rot=[1 0 0;0 1 0;0 0 1]  CS5Pos=[-0.0179146 0.0277141 0.0258426]  CS5Rot=[1 0 0;0 1 0;0 0 1]  CS6Pos=[0.0480334 0.0678885 0.0433426]  CS6Rot=[1 0 0;0 1 0;0 0 1]  CS7Pos=[]  CS7Rot=[]  CS8Pos=[]  CS8Rot=[]  CS9Pos=[]  CS9Rot=[]  CS10Pos=[]  CS10Rot=[]  CS11Pos=[]  CS11Rot=[]  CS12Pos=[]  CS12Rot=[]  CS13Pos=[]  CS13Rot=[]  CS14Pos=[]  CS14Rot=[]  CS15Pos=[]  CS15Rot=[]  CS16Pos=[]  CS16Rot=[]  CS17Pos=[]  CS17Rot=[]  CS18Pos=[]  CS18Rot=[]  CS19Pos=[]  CS19Rot=[]  CS20Pos=[]  CS20Rot=[]
  link3-2 : mblibv1/Bodies/Body  LConnTagsString=CS2|CS6  RConnTagsString=CS3|CS4|CS5  UpdateFromCAD=on  PMImportedID=link3-2  DialogClass=MechanicalBodyBlock  Mass=0.0131167  MassUnits=kg  InertiaUnits=kg*m^2  Inertia=[7.39603e-06,-4.27092e-06,-1.73808e-08;-4.27092e-06,6.72647e-06,-1.85249e-08;-1.73808e-08,-1.85249e-08,1.01055e-05]  Shape=Cylinder  ShapeDims=[1 1]  ShapeUnits=m  ShapeUse=false  Density=1  DensityUnits=kg/m^3  DensityUse=false  GraphicsMode=GFXFILE  GraphicsFileName=GripperForSimulink - link3-2.STL  BodyColorSelMode=COLORPALETTE  BodyColor=[0.792157;0.819608;0.933333]  AttachedToCS=CS1  CG=Right$CG$[0.0128329 -0.0582585 0.0232454]$WORLD$WORLD$m$[0.944391 0.328825 0;0.328825 -0.944391 0;0 0 -1]$3x3 Transform$rad$WORLD$false$link3-2::CG(AUTOGEN)  WorkingFrames=Right$CS1$[-0.0214827 -0.0304467 0.0258426]$WORLD$WORLD$m$[0.944391 0.328825 0;0.328825 -0.944391 0;0 0 -1]$3x3 Transform$rad$WORLD$false$link3-2::CS1(AUTOGEN)#Left$CS2$[-0.00973859 -0.0630284 0.0358426]$WORLD$WORLD$m$[1 0 0;0 1 0;0 0 1]$3x3 Transform$rad$WORLD$true$base-1:-:link3-2::link3-2(AUTOGEN)#Right$CS3$[0.0480334 -0.0694542 0.0483426]$WORLD$WORLD$m$[1 0 0;0 1 0;0 0 1]$3x3 Transform$rad$WORLD$true$grip-2:-:link3-2::link3-2(AUTOGEN)#Right$CS4$[-0.0179146 -0.0292797 0.0208426]$WORLD$WORLD$m$[1 0 0;0 1 0;0 0 1]$3x3 Transform$rad$WORLD$true$link3-2:-:pin15mm-4::link3-2(AUTOGEN)#Right$CS5$[0.0480334 -0.0694542 0.0483426]$WORLD$WORLD$m$[1 0 0;0 1 0;0 0 1]$3x3 Transform$rad$WORLD$true$link3-2:-:pin50mm-2::link3-2(AUTOGEN)#Left$CS6$[-0.0179146 -0.0292797 0.0208426]$WORLD$WORLD$m$[1 0 0;0 1 0;0 0 1]$3x3 Transform$rad$WORLD$true$link1-2:-:link3-2::link3-2(AUTOGEN)  CGPos=[0.0128329 -0.0582585 0.0232454]  CGRot=[0.944391 0.328825 0;0.328825 -0.944391 0;0 0 -1]  CS0Pos=[]  CS0Rot=[]  CS1Pos=[-0.0214827 -0.0304467 0.0258426]  CS1Rot=[0.944391 0.328825 0;0.328825 -0.944391 0;0 0 -1]  CS2Pos=[-0.00973859 -0.0630284 0.0358426]  CS2Rot=[1 0 0;0 1 0;0 0 1]  CS3Pos=[0.0480334 -0.0694542 0.0483426]  CS3Rot=[1 0 0;0 1 0;0 0 1]  CS4Pos=[-0.0179146 -0.0292797 0.0208426]  CS4Rot=[1 0 0;0 1 0;0 0 1]  CS5Pos=[0.0480334 -0.0694542 0.0483426]  CS5Rot=[1 0 0;0 1 0;0 0 1]  CS6Pos=[-0.0179146 -0.0292797 0.0208426]  CS6Rot=[1 0 0;0 1 0;0 0 1]  CS7Pos=[]  CS7Rot=[]  CS8Pos=[]  CS8Rot=[]  CS9Pos=[]  CS9Rot=[]  CS10Pos=[]  CS10Rot=[]  CS11Pos=[]  CS11Rot=[]  CS12Pos=[]  CS12Rot=[]  CS13Pos=[]  CS13Rot=[]  CS14Pos=[]  CS14Rot=[]  CS15Pos=[]  CS15Rot=[]  CS16Pos=[]  CS16Rot=[]  CS17Pos=[]  CS17Rot=[]  CS18Pos=[]  CS18Rot=[]  CS19Pos=[]  CS19Rot=[]  CS20Pos=[]  CS20Rot=[]
  link4-1 : mblibv1/Bodies/Body  LConnTagsString=CS2|CS3  RConnTagsString=CS4|CS5|CS6|CS7  UpdateFromCAD=on  PMImportedID=link4-1  DialogClass=MechanicalBodyBlock  Mass=0.0188094  MassUnits=kg  InertiaUnits=kg*m^2  Inertia=[5.2882e-06,0,0;0,1.73698e-06,0;0,0,5.12283e-06]  Shape=Cylinder  ShapeDims=[1 1]  ShapeUnits=m  ShapeUse=false  Density=1  DensityUnits=kg/m^3  DensityUse=false  GraphicsMode=GFXFILE  GraphicsFileName=GripperForSimulink - link4-1.STL  BodyColorSelMode=COLORPALETTE  BodyColor=[0.792157;0.819608;0.933333]  AttachedToCS=CS1  CG=Right$CG$[-0.0378581 -0.000782836 0.0233426]$WORLD$WORLD$m$[1 0 0;0 1 0;0 0 1]$3x3 Transform$rad$WORLD$false$link4-1::CG(AUTOGEN)  WorkingFrames=Right$CS1$[-0.0378581 -0.000782836 0.0108426]$WORLD$WORLD$m$[1 0 0;0 1 0;0 0 1]$3x3 Transform$rad$WORLD$false$link4-1::CS1(AUTOGEN)#Left$CS2$[0.0165606 -0.000782836 0.0233426]$WORLD$WORLD$m$[1 0 0;0 1 0;0 0 1]$3x3 Transform$rad$WORLD$true$base-1:-:link4-1::link4-1(AUTOGEN)#Left$CS3$[-0.0378581 0.0292172 0.0208426]$WORLD$WORLD$m$[1 0 0;0 1 0;0 0 1]$3x3 Transform$rad$WORLD$true$link1-1:-:link4-1::link4-1(AUTOGEN)#Right$CS4$[-0.0378581 0.0292172 0.0108426]$WORLD$WORLD$m$[1 0 0;0 1 0;0 0 1]$3x3 Transform$rad$WORLD$true$link4-1:-:pin15mm-1::link4-1(AUTOGEN)#Right$CS5$[-0.0378581 -0.0307828 0.0108426]$WORLD$WORLD$m$[1 0 0;0 1 0;0 0 1]$3x3 Transform$rad$WORLD$true$link4-1:-:pin15mm-3::link4-1(AUTOGEN)#Right$CS6$[-0.0253581 -0.0132828 0.0358426]$WORLD$WORLD$m$[1 0 0;0 1 0;0 0 1]$3x3 Transform$rad$WORLD$true$driveshaft-2:-:link4-1::link4-1(AUTOGEN)#Right$CS7$[-0.0378581 -0.0307828 0.0108426]$WORLD$WORLD$m$[1 0 0;0 1 0;0 0 1]$3x3 Transform$rad$WORLD$true$link1-2:-:link4-1::link4-1(AUTOGEN)  CGPos=[-0.0378581 -0.000782836 0.0233426]  CGRot=[1 0 0;0 1 0;0 0 1]  CS0Pos=[]  CS0Rot=[]  CS1Pos=[-0.0378581 -0.000782836 0.0108426]  CS1Rot=[1 0 0;0 1 0;0 0 1]  CS2Pos=[0.0165606 -0.000782836 0.0233426]  CS2Rot=[1 0 0;0 1 0;0 0 1]  CS3Pos=[-0.0378581 0.0292172 0.0208426]  CS3Rot=[1 0 0;0 1 0;0 0 1]  CS4Pos=[-0.0378581 0.0292172 0.0108426]  CS4Rot=[1 0 0;0 1 0;0 0 1]  CS5Pos=[-0.0378581 -0.0307828 0.0108426]  CS5Rot=[1 0 0;0 1 0;0 0 1]  CS6Pos=[-0.0253581 -0.0132828 0.0358426]  CS6Rot=[1 0 0;0 1 0;0 0 1]  CS7Pos=[-0.0378581 -0.0307828 0.0108426]  CS7Rot=[1 0 0;0 1 0;0 0 1]  CS8Pos=[]  CS8Rot=[]  CS9Pos=[]  CS9Rot=[]  CS10Pos=[]  CS10Rot=[]  CS11Pos=[]  CS11Rot=[]  CS12Pos=[]  CS12Rot=[]  CS13Pos=[]  CS13Rot=[]  CS14Pos=[]  CS14Rot=[]  CS15Pos=[]  CS15Rot=[]  CS16Pos=[]  CS16Rot=[]  CS17Pos=[]  CS17Rot=[]  CS18Pos=[]  CS18Rot=[]  CS19Pos=[]  CS19Rot=[]  CS20Pos=[]  CS20Rot=[]
  pin1-2 : mblibv1/Bodies/Body  LConnTagsString=CS2  UpdateFromCAD=on  PMImportedID=pin1-2  DialogClass=MechanicalBodyBlock  Mass=0.00200043  MassUnits=kg  InertiaUnits=kg*m^2  Inertia=[2.7207e-07,0,0;0,1.59386e-08,0;0,0,2.7207e-07]  Shape=Cylinder  ShapeDims=[1 1]  ShapeUnits=m  ShapeUse=false  Density=1  DensityUnits=kg/m^3  DensityUse=false  GraphicsMode=GFXFILE  GraphicsFileName=GripperForSimulink - pin1-2.STL  BodyColorSelMode=COLORPALETTE  BodyColor=[0.666667;0.698039;0.768627]  AttachedToCS=CS1  CG=Right$CG$[-0.00973859 0.0614627 0.0230926]$WORLD$WORLD$m$[-0.156349 0 -0.987702;0.987702 0 -0.156349;0 -1 0]$3x3 Transform$rad$WORLD$false$pin1-2::CG(AUTOGEN)  WorkingFrames=Right$CS1$[-0.00973859 0.0614627 0.0430926]$WORLD$WORLD$m$[-0.156349 0 -0.987702;0.987702 0 -0.156349;0 -1 0]$3x3 Transform$rad$WORLD$false$pin1-2::CS1(AUTOGEN)#Left$CS2$[-0.00973859 0.0614627 0.0108426]$WORLD$WORLD$m$[1 0 0;0 1 0;0 0 1]$3x3 Transform$rad$WORLD$true$base-1:-:pin1-2::pin1-2(AUTOGEN)  CGPos=[-0.00973859 0.0614627 0.0230926]  CGRot=[-0.156349 0 -0.987702;0.987702 0 -0.156349;0 -1 0]  CS0Pos=[]  CS0Rot=[]  CS1Pos=[-0.00973859 0.0614627 0.0430926]  CS1Rot=[-0.156349 0 -0.987702;0.987702 0 -0.156349;0 -1 0]  CS2Pos=[-0.00973859 0.0614627 0.0108426]  CS2Rot=[1 0 0;0 1 0;0 0 1]  CS3Pos=[]  CS3Rot=[]  CS4Pos=[]  CS4Rot=[]  CS5Pos=[]  CS5Rot=[]  CS6Pos=[]  CS6Rot=[]  CS7Pos=[]  CS7Rot=[]  CS8Pos=[]  CS8Rot=[]  CS9Pos=[]  CS9Rot=[]  CS10Pos=[]  CS10Rot=[]  CS11Pos=[]  CS11Rot=[]  CS12Pos=[]  CS12Rot=[]  CS13Pos=[]  CS13Rot=[]  CS14Pos=[]  CS14Rot=[]  CS15Pos=[]  CS15Rot=[]  CS16Pos=[]  CS16Rot=[]  CS17Pos=[]  CS17Rot=[]  CS18Pos=[]  CS18Rot=[]  CS19Pos=[]  CS19Rot=[]  CS20Pos=[]  CS20Rot=[]
  pin1-5 : mblibv1/Bodies/Body  LConnTagsString=CS2  UpdateFromCAD=on  PMImportedID=pin1-5  DialogClass=MechanicalBodyBlock  Mass=0.00200043  MassUnits=kg  InertiaUnits=kg*m^2  Inertia=[2.7207e-07,0,0;0,1.59386e-08,0;0,0,2.7207e-07]  Shape=Cylinder  ShapeDims=[1 1]  ShapeUnits=m  ShapeUse=false  Density=1  DensityUnits=kg/m^3  DensityUse=false  GraphicsMode=GFXFILE  GraphicsFileName=GripperForSimulink - pin1-5.STL  BodyColorSelMode=COLORPALETTE  BodyColor=[0.666667;0.698039;0.768627]  AttachedToCS=CS1  CG=Right$CG$[-0.00973859 -0.0630284 0.0230926]$WORLD$WORLD$m$[1 0 0;0 0 -1;0 1 0]$3x3 Transform$rad$WORLD$false$pin1-5::CG(AUTOGEN)  WorkingFrames=Right$CS1$[-0.00973859 -0.0630284 0.00309264]$WORLD$WORLD$m$[1 0 0;0 0 -1;0 1 0]$3x3 Transform$rad$WORLD$false$pin1-5::CS1(AUTOGEN)#Left$CS2$[-0.00973859 -0.0630284 0.0358426]$WORLD$WORLD$m$[1 0 0;0 1 0;0 0 1]$3x3 Transform$rad$WORLD$true$base-1:-:pin1-5::pin1-5(AUTOGEN)  CGPos=[-0.00973859 -0.0630284 0.0230926]  CGRot=[1 0 0;0 0 -1;0 1 0]  CS0Pos=[]  CS0Rot=[]  CS1Pos=[-0.00973859 -0.0630284 0.00309264]  CS1Rot=[1 0 0;0 0 -1;0 1 0]  CS2Pos=[-0.00973859 -0.0630284 0.0358426]  CS2Rot=[1 0 0;0 1 0;0 0 1]  CS3Pos=[]  CS3Rot=[]  CS4Pos=[]  CS4Rot=[]  CS5Pos=[]  CS5Rot=[]  CS6Pos=[]  CS6Rot=[]  CS7Pos=[]  CS7Rot=[]  CS8Pos=[]  CS8Rot=[]  CS9Pos=[]  CS9Rot=[]  CS10Pos=[]  CS10Rot=[]  CS11Pos=[]  CS11Rot=[]  CS12Pos=[]  CS12Rot=[]  CS13Pos=[]  CS13Rot=[]  CS14Pos=[]  CS14Rot=[]  CS15Pos=[]  CS15Rot=[]  CS16Pos=[]  CS16Rot=[]  CS17Pos=[]  CS17Rot=[]  CS18Pos=[]  CS18Rot=[]  CS19Pos=[]  CS19Rot=[]  CS20Pos=[]  CS20Rot=[]
  pin15mm-1 : mblibv1/Bodies/Body  LConnTagsString=CS2  UpdateFromCAD=on  PMImportedID=pin15mm-1  DialogClass=MechanicalBodyBlock  Mass=0.000743798  MassUnits=kg  InertiaUnits=kg*m^2  Inertia=[1.65411e-08,0,0;0,1.65411e-08,0;0,0,5.88554e-09]  Shape=Cylinder  ShapeDims=[1 1]  ShapeUnits=m  ShapeUse=false  Density=1  DensityUnits=kg/m^3  DensityUse=false  GraphicsMode=GFXFILE  GraphicsFileName=GripperForSimulink - pin15mm-1.STL  BodyColorSelMode=COLORPALETTE  BodyColor=[0.666667;0.698039;0.768627]  AttachedToCS=CS1  CG=Right$CG$[-0.0378581 0.0292172 0.0233426]$WORLD$WORLD$m$[1 0 0;0 1 0;0 0 1]$3x3 Transform$rad$WORLD$false$pin15mm-1::CG(AUTOGEN)  WorkingFrames=Right$CS1$[-0.0378581 0.0292172 0.0158426]$WORLD$WORLD$m$[1 0 0;0 1 0;0 0 1]$3x3 Transform$rad$WORLD$false$pin15mm-1::CS1(AUTOGEN)#Left$CS2$[-0.0378581 0.0292172 0.0108426]$WORLD$WORLD$m$[1 0 0;0 1 0;0 0 1]$3x3 Transform$rad$WORLD$true$link4-1:-:pin15mm-1::pin15mm-1(AUTOGEN)  CGPos=[-0.0378581 0.0292172 0.0233426]  CGRot=[1 0 0;0 1 0;0 0 1]  CS0Pos=[]  CS0Rot=[]  CS1Pos=[-0.0378581 0.0292172 0.0158426]  CS1Rot=[1 0 0;0 1 0;0 0 1]  CS2Pos=[-0.0378581 0.0292172 0.0108426]  CS2Rot=[1 0 0;0 1 0;0 0 1]  CS3Pos=[]  CS3Rot=[]  CS4Pos=[]  CS4Rot=[]  CS5Pos=[]  CS5Rot=[]  CS6Pos=[]  CS6Rot=[]  CS7Pos=[]  CS7Rot=[]  CS8Pos=[]  CS8Rot=[]  CS9Pos=[]  CS9Rot=[]  CS10Pos=[]  CS10Rot=[]  CS11Pos=[]  CS11Rot=[]  CS12Pos=[]  CS12Rot=[]  CS13Pos=[]  CS13Rot=[]  CS14Pos=[]  CS14Rot=[]  CS15Pos=[]  CS15Rot=[]  CS16Pos=[]  CS16Rot=[]  CS17Pos=[]  CS17Rot=[]  CS18Pos=[]  CS18Rot=[]  CS19Pos=[]  CS19Rot=[]  CS20Pos=[]  CS20Rot=[]
  pin15mm-2 : mblibv1/Bodies/Body  LConnTagsString=CS2  UpdateFromCAD=on  PMImportedID=pin15mm-2  DialogClass=MechanicalBodyBlock  Mass=0.000743798  MassUnits=kg  InertiaUnits=kg*m^2  Inertia=[1.65411e-08,0,0;0,1.65411e-08,0;0,0,5.88554e-09]  Shape=Cylinder  ShapeDims=[1 1]  ShapeUnits=m  ShapeUse=false  Density=1  DensityUnits=kg/m^3  DensityUse=false  GraphicsMode=GFXFILE  GraphicsFileName=GripperForSimulink - pin15mm-2.STL  BodyColorSelMode=COLORPALETTE  BodyColor=[0.666667;0.698039;0.768627]  AttachedToCS=CS1  CG=Right$CG$[-0.0179146 0.0277141 0.0233426]$WORLD$WORLD$m$[1 0 0;0 1 0;0 0 1]$3x3 Transform$rad$WORLD$false$pin15mm-2::CG(AUTOGEN)  WorkingFrames=Right$CS1$[-0.0179146 0.0277141 0.0158426]$WORLD$WORLD$m$[1 0 0;0 1 0;0 0 1]$3x3 Transform$rad$WORLD$false$pin15mm-2::CS1(AUTOGEN)#Left$CS2$[-0.0179146 0.0277141 0.0258426]$WORLD$WORLD$m$[1 0 0;0 1 0;0 0 1]$3x3 Transform$rad$WORLD$true$link3-1:-:pin15mm-2::pin15mm-2(AUTOGEN)  CGPos=[-0.0179146 0.0277141 0.0233426]  CGRot=[1 0 0;0 1 0;0 0 1]  CS0Pos=[]  CS0Rot=[]  CS1Pos=[-0.0179146 0.0277141 0.0158426]  CS1Rot=[1 0 0;0 1 0;0 0 1]  CS2Pos=[-0.0179146 0.0277141 0.0258426]  CS2Rot=[1 0 0;0 1 0;0 0 1]  CS3Pos=[]  CS3Rot=[]  CS4Pos=[]  CS4Rot=[]  CS5Pos=[]  CS5Rot=[]  CS6Pos=[]  CS6Rot=[]  CS7Pos=[]  CS7Rot=[]  CS8Pos=[]  CS8Rot=[]  CS9Pos=[]  CS9Rot=[]  CS10Pos=[]  CS10Rot=[]  CS11Pos=[]  CS11Rot=[]  CS12Pos=[]  CS12Rot=[]  CS13Pos=[]  CS13Rot=[]  CS14Pos=[]  CS14Rot=[]  CS15Pos=[]  CS15Rot=[]  CS16Pos=[]  CS16Rot=[]  CS17Pos=[]  CS17Rot=[]  CS18Pos=[]  CS18Rot=[]  CS19Pos=[]  CS19Rot=[]  CS20Pos=[]  CS20Rot=[]
  pin15mm-3 : mblibv1/Bodies/Body  LConnTagsString=CS2  UpdateFromCAD=on  PMImportedID=pin15mm-3  DialogClass=MechanicalBodyBlock  Mass=0.000743798  MassUnits=kg  InertiaUnits=kg*m^2  Inertia=[1.65411e-08,0,0;0,1.65411e-08,0;0,0,5.88554e-09]  Shape=Cylinder  ShapeDims=[1 1]  ShapeUnits=m  ShapeUse=false  Density=1  DensityUnits=kg/m^3  DensityUse=false  GraphicsMode=GFXFILE  GraphicsFileName=GripperForSimulink - pin15mm-3.STL  BodyColorSelMode=COLORPALETTE  BodyColor=[0.666667;0.698039;0.768627]  AttachedToCS=CS1  CG=Right$CG$[-0.0378581 -0.0307828 0.0233426]$WORLD$WORLD$m$[1 0 0;0 1 0;0 0 1]$3x3 Transform$rad$WORLD$false$pin15mm-3::CG(AUTOGEN)  WorkingFrames=Right$CS1$[-0.0378581 -0.0307828 0.0158426]$WORLD$WORLD$m$[1 0 0;0 1 0;0 0 1]$3x3 Transform$rad$WORLD$false$pin15mm-3::CS1(AUTOGEN)#Left$CS2$[-0.0378581 -0.0307828 0.0108426]$WORLD$WORLD$m$[1 0 0;0 1 0;0 0 1]$3x3 Transform$rad$WORLD$true$link4-1:-:pin15mm-3::pin15mm-3(AUTOGEN)  CGPos=[-0.0378581 -0.0307828 0.0233426]  CGRot=[1 0 0;0 1 0;0 0 1]  CS0Pos=[]  CS0Rot=[]  CS1Pos=[-0.0378581 -0.0307828 0.0158426]  CS1Rot=[1 0 0;0 1 0;0 0 1]  CS2Pos=[-0.0378581 -0.0307828 0.0108426]  CS2Rot=[1 0 0;0 1 0;0 0 1]  CS3Pos=[]  CS3Rot=[]  CS4Pos=[]  CS4Rot=[]  CS5Pos=[]  CS5Rot=[]  CS6Pos=[]  CS6Rot=[]  CS7Pos=[]  CS7Rot=[]  CS8Pos=[]  CS8Rot=[]  CS9Pos=[]  CS9Rot=[]  CS10Pos=[]  CS10Rot=[]  CS11Pos=[]  CS11Rot=[]  CS12Pos=[]  CS12Rot=[]  CS13Pos=[]  CS13Rot=[]  CS14Pos=[]  CS14Rot=[]  CS15Pos=[]  CS15Rot=[]  CS16Pos=[]  CS16Rot=[]  CS17Pos=[]  CS17Rot=[]  CS18Pos=[]  CS18Rot=[]  CS19Pos=[]  CS19Rot=[]  CS20Pos=[]  CS20Rot=[]
  pin15mm-4 : mblibv1/Bodies/Body  LConnTagsString=CS2  UpdateFromCAD=on  PMImportedID=pin15mm-4  DialogClass=MechanicalBodyBlock  Mass=0.000743798  MassUnits=kg  InertiaUnits=kg*m^2  Inertia=[1.65411e-08,0,0;0,1.65411e-08,0;0,0,5.88554e-09]  Shape=Cylinder  ShapeDims=[1 1]  ShapeUnits=m  ShapeUse=false  Density=1  DensityUnits=kg/m^3  DensityUse=false  GraphicsMode=GFXFILE  GraphicsFileName=GripperForSimulink - pin15mm-4.STL  BodyColorSelMode=COLORPALETTE  BodyColor=[0.666667;0.698039;0.768627]  AttachedToCS=CS1  CG=Right$CG$[-0.0179146 -0.0292797 0.0233426]$WORLD$WORLD$m$[1 0 0;0 1 0;0 0 1]$3x3 Transform$rad$WORLD$false$pin15mm-4::CG(AUTOGEN)  WorkingFrames=Right$CS1$[-0.0179146 -0.0292797 0.0158426]$WORLD$WORLD$m$[1 0 0;0 1 0;0 0 1]$3x3 Transform$rad$WORLD$false$pin15mm-4::CS1(AUTOGEN)#Left$CS2$[-0.0179146 -0.0292797 0.0208426]$WORLD$WORLD$m$[1 0 0;0 1 0;0 0 1]$3x3 Transform$rad$WORLD$true$link3-2:-:pin15mm-4::pin15mm-4(AUTOGEN)  CGPos=[-0.0179146 -0.0292797 0.0233426]  CGRot=[1 0 0;0 1 0;0 0 1]  CS0Pos=[]  CS0Rot=[]  CS1Pos=[-0.0179146 -0.0292797 0.0158426]  CS1Rot=[1 0 0;0 1 0;0 0 1]  CS2Pos=[-0.0179146 -0.0292797 0.0208426]  CS2Rot=[1 0 0;0 1 0;0 0 1]  CS3Pos=[]  CS3Rot=[]  CS4Pos=[]  CS4Rot=[]  CS5Pos=[]  CS5Rot=[]  CS6Pos=[]  CS6Rot=[]  CS7Pos=[]  CS7Rot=[]  CS8Pos=[]  CS8Rot=[]  CS9Pos=[]  CS9Rot=[]  CS10Pos=[]  CS10Rot=[]  CS11Pos=[]  CS11Rot=[]  CS12Pos=[]  CS12Rot=[]  CS13Pos=[]  CS13Rot=[]  CS14Pos=[]  CS14Rot=[]  CS15Pos=[]  CS15Rot=[]  CS16Pos=[]  CS16Rot=[]  CS17Pos=[]  CS17Rot=[]  CS18Pos=[]  CS18Rot=[]  CS19Pos=[]  CS19Rot=[]  CS20Pos=[]  CS20Rot=[]
  pin50mm-1 : mblibv1/Bodies/Body  LConnTagsString=CS3  RConnTagsString=CS2  UpdateFromCAD=on  PMImportedID=pin50mm-1  DialogClass=MechanicalBodyBlock  Mass=0.00250309  MassUnits=kg  InertiaUnits=kg*m^2  Inertia=[5.27329e-07,0,0;0,5.27329e-07,0;0,0,1.99599e-08]  Shape=Cylinder  ShapeDims=[1 1]  ShapeUnits=m  ShapeUse=false  Density=1  DensityUnits=kg/m^3  DensityUse=false  GraphicsMode=GFXFILE  GraphicsFileName=GripperForSimulink - pin50mm-1.STL  BodyColorSelMode=COLORPALETTE  BodyColor=[0.666667;0.698039;0.768627]  AttachedToCS=CS1  CG=Right$CG$[0.00656063 -0.0378305 0.0233426]$WORLD$WORLD$m$[1 0 0;0 1 0;0 0 1]$3x3 Transform$rad$WORLD$false$pin50mm-1::CG(AUTOGEN)  WorkingFrames=Right$CS1$[0.00656063 -0.0378305 -0.00165736]$WORLD$WORLD$m$[1 0 0;0 1 0;0 0 1]$3x3 Transform$rad$WORLD$false$pin50mm-1::CS1(AUTOGEN)#Right$CS2$[0.00656063 -0.0378305 0.0483426]$WORLD$WORLD$m$[1 0 0;0 1 0;0 0 1]$3x3 Transform$rad$WORLD$true$link2-4:-:pin50mm-1::pin50mm-1(AUTOGEN)#Left$CS3$[0.00656063 -0.0378305 0.0433426]$WORLD$WORLD$m$[1 0 0;0 1 0;0 0 1]$3x3 Transform$rad$WORLD$true$link2-2:-:pin50mm-1::pin50mm-1(AUTOGEN)  CGPos=[0.00656063 -0.0378305 0.0233426]  CGRot=[1 0 0;0 1 0;0 0 1]  CS0Pos=[]  CS0Rot=[]  CS1Pos=[0.00656063 -0.0378305 -0.00165736]  CS1Rot=[1 0 0;0 1 0;0 0 1]  CS2Pos=[0.00656063 -0.0378305 0.0483426]  CS2Rot=[1 0 0;0 1 0;0 0 1]  CS3Pos=[0.00656063 -0.0378305 0.0433426]  CS3Rot=[1 0 0;0 1 0;0 0 1]  CS4Pos=[]  CS4Rot=[]  CS5Pos=[]  CS5Rot=[]  CS6Pos=[]  CS6Rot=[]  CS7Pos=[]  CS7Rot=[]  CS8Pos=[]  CS8Rot=[]  CS9Pos=[]  CS9Rot=[]  CS10Pos=[]  CS10Rot=[]  CS11Pos=[]  CS11Rot=[]  CS12Pos=[]  CS12Rot=[]  CS13Pos=[]  CS13Rot=[]  CS14Pos=[]  CS14Rot=[]  CS15Pos=[]  CS15Rot=[]  CS16Pos=[]  CS16Rot=[]  CS17Pos=[]  CS17Rot=[]  CS18Pos=[]  CS18Rot=[]  CS19Pos=[]  CS19Rot=[]  CS20Pos=[]  CS20Rot=[]
  pin50mm-2 : mblibv1/Bodies/Body  LConnTagsString=CS2  UpdateFromCAD=on  PMImportedID=pin50mm-2  DialogClass=MechanicalBodyBlock  Mass=0.00250309  MassUnits=kg  InertiaUnits=kg*m^2  Inertia=[5.27329e-07,0,0;0,5.27329e-07,0;0,0,1.99599e-08]  Shape=Cylinder  ShapeDims=[1 1]  ShapeUnits=m  ShapeUse=false  Density=1  DensityUnits=kg/m^3  DensityUse=false  GraphicsMode=GFXFILE  GraphicsFileName=GripperForSimulink - pin50mm-2.STL  BodyColorSelMode=COLORPALETTE  BodyColor=[0.666667;0.698039;0.768627]  AttachedToCS=CS1  CG=Right$CG$[0.0480334 -0.0694542 0.0233426]$WORLD$WORLD$m$[1 0 0;0 1 0;0 0 1]$3x3 Transform$rad$WORLD$false$pin50mm-2::CG(AUTOGEN)  WorkingFrames=Right$CS1$[0.0480334 -0.0694542 -0.00165736]$WORLD$WORLD$m$[1 0 0;0 1 0;0 0 1]$3x3 Transform$rad$WORLD$false$pin50mm-2::CS1(AUTOGEN)#Left$CS2$[0.0480334 -0.0694542 0.0483426]$WORLD$WORLD$m$[1 0 0;0 1 0;0 0 1]$3x3 Transform$rad$WORLD$true$link3-2:-:pin50mm-2::pin50mm-2(AUTOGEN)  CGPos=[0.0480334 -0.0694542 0.0233426]  CGRot=[1 0 0;0 1 0;0 0 1]  CS0Pos=[]  CS0Rot=[]  CS1Pos=[0.0480334 -0.0694542 -0.00165736]  CS1Rot=[1 0 0;0 1 0;0 0 1]  CS2Pos=[0.0480334 -0.0694542 0.0483426]  CS2Rot=[1 0 0;0 1 0;0 0 1]  CS3Pos=[]  CS3Rot=[]  CS4Pos=[]  CS4Rot=[]  CS5Pos=[]  CS5Rot=[]  CS6Pos=[]  CS6Rot=[]  CS7Pos=[]  CS7Rot=[]  CS8Pos=[]  CS8Rot=[]  CS9Pos=[]  CS9Rot=[]  CS10Pos=[]  CS10Rot=[]  CS11Pos=[]  CS11Rot=[]  CS12Pos=[]  CS12Rot=[]  CS13Pos=[]  CS13Rot=[]  CS14Pos=[]  CS14Rot=[]  CS15Pos=[]  CS15Rot=[]  CS16Pos=[]  CS16Rot=[]  CS17Pos=[]  CS17Rot=[]  CS18Pos=[]  CS18Rot=[]  CS19Pos=[]  CS19Rot=[]  CS20Pos=[]  CS20Rot=[]
  pin50mm-3 : mblibv1/Bodies/Body  LConnTagsString=CS3  RConnTagsString=CS2  UpdateFromCAD=on  PMImportedID=pin50mm-3  DialogClass=MechanicalBodyBlock  Mass=0.00250309  MassUnits=kg  InertiaUnits=kg*m^2  Inertia=[5.27329e-07,0,0;0,5.27329e-07,0;0,0,1.99599e-08]  Shape=Cylinder  ShapeDims=[1 1]  ShapeUnits=m  ShapeUse=false  Density=1  DensityUnits=kg/m^3  DensityUse=false  GraphicsMode=GFXFILE  GraphicsFileName=GripperForSimulink - pin50mm-3.STL  BodyColorSelMode=COLORPALETTE  BodyColor=[0.666667;0.698039;0.768627]  AttachedToCS=CS1  CG=Right$CG$[0.0560713 -0.0448086 0.0233426]$WORLD$WORLD$m$[1 0 0;0 1 0;0 0 1]$3x3 Transform$rad$WORLD$false$pin50mm-3::CG(AUTOGEN)  WorkingFrames=Right$CS1$[0.0560713 -0.0448086 -0.00165736]$WORLD$WORLD$m$[1 0 0;0 1 0;0 0 1]$3x3 Transform$rad$WORLD$false$pin50mm-3::CS1(AUTOGEN)#Right$CS2$[0.0560713 -0.0448086 0.0483426]$WORLD$WORLD$m$[1 0 0;0 1 0;0 0 1]$3x3 Transform$rad$WORLD$true$link2-4:-:pin50mm-3::pin50mm-3(AUTOGEN)#Left$CS3$[0.0560713 -0.0448086 0.0433426]$WORLD$WORLD$m$[1 0 0;0 1 0;0 0 1]$3x3 Transform$rad$WORLD$true$link2-2:-:pin50mm-3::pin50mm-3(AUTOGEN)  CGPos=[0.0560713 -0.0448086 0.0233426]  CGRot=[1 0 0;0 1 0;0 0 1]  CS0Pos=[]  CS0Rot=[]  CS1Pos=[0.0560713 -0.0448086 -0.00165736]  CS1Rot=[1 0 0;0 1 0;0 0 1]  CS2Pos=[0.0560713 -0.0448086 0.0483426]  CS2Rot=[1 0 0;0 1 0;0 0 1]  CS3Pos=[0.0560713 -0.0448086 0.0433426]  CS3Rot=[1 0 0;0 1 0;0 0 1]  CS4Pos=[]  CS4Rot=[]  CS5Pos=[]  CS5Rot=[]  CS6Pos=[]  CS6Rot=[]  CS7Pos=[]  CS7Rot=[]  CS8Pos=[]  CS8Rot=[]  CS9Pos=[]  CS9Rot=[]  CS10Pos=[]  CS10Rot=[]  CS11Pos=[]  CS11Rot=[]  CS12Pos=[]  CS12Rot=[]  CS13Pos=[]  CS13Rot=[]  CS14Pos=[]  CS14Rot=[]  CS15Pos=[]  CS15Rot=[]  CS16Pos=[]  CS16Rot=[]  CS17Pos=[]  CS17Rot=[]  CS18Pos=[]  CS18Rot=[]  CS19Pos=[]  CS19Rot=[]  CS20Pos=[]  CS20Rot=[]
  pin50mm-4 : mblibv1/Bodies/Body  RConnTagsString=CS2  UpdateFromCAD=on  PMImportedID=pin50mm-4  DialogClass=MechanicalBodyBlock  Mass=0.00250309  MassUnits=kg  InertiaUnits=kg*m^2  Inertia=[5.27329e-07,0,0;0,5.27329e-07,0;0,0,1.99599e-08]  Shape=Cylinder  ShapeDims=[1 1]  ShapeUnits=m  ShapeUse=false  Density=1  DensityUnits=kg/m^3  DensityUse=false  GraphicsMode=GFXFILE  GraphicsFileName=GripperForSimulink - pin50mm-4.STL  BodyColorSelMode=COLORPALETTE  BodyColor=[0.666667;0.698039;0.768627]  AttachedToCS=CS1  CG=Right$CG$[0.00656063 0.0362648 0.0235926]$WORLD$WORLD$m$[1 0 0;0 1 0;0 0 1]$3x3 Transform$rad$WORLD$false$pin50mm-4::CG(AUTOGEN)  WorkingFrames=Right$CS1$[0.00656063 0.0362648 -0.00140736]$WORLD$WORLD$m$[1 0 0;0 1 0;0 0 1]$3x3 Transform$rad$WORLD$false$pin50mm-4::CS1(AUTOGEN)#Right$CS2$[0.00656063 0.0362648 0.0485926]$WORLD$WORLD$m$[1 0 0;0 1 0;0 0 1]$3x3 Transform$rad$WORLD$true$link2-3:-:pin50mm-4::pin50mm-4(AUTOGEN)  CGPos=[0.00656063 0.0362648 0.0235926]  CGRot=[1 0 0;0 1 0;0 0 1]  CS0Pos=[]  CS0Rot=[]  CS1Pos=[0.00656063 0.0362648 -0.00140736]  CS1Rot=[1 0 0;0 1 0;0 0 1]  CS2Pos=[0.00656063 0.0362648 0.0485926]  CS2Rot=[1 0 0;0 1 0;0 0 1]  CS3Pos=[]  CS3Rot=[]  CS4Pos=[]  CS4Rot=[]  CS5Pos=[]  CS5Rot=[]  CS6Pos=[]  CS6Rot=[]  CS7Pos=[]  CS7Rot=[]  CS8Pos=[]  CS8Rot=[]  CS9Pos=[]  CS9Rot=[]  CS10Pos=[]  CS10Rot=[]  CS11Pos=[]  CS11Rot=[]  CS12Pos=[]  CS12Rot=[]  CS13Pos=[]  CS13Rot=[]  CS14Pos=[]  CS14Rot=[]  CS15Pos=[]  CS15Rot=[]  CS16Pos=[]  CS16Rot=[]  CS17Pos=[]  CS17Rot=[]  CS18Pos=[]  CS18Rot=[]  CS19Pos=[]  CS19Rot=[]  CS20Pos=[]  CS20Rot=[]
  pin50mm-5 : mblibv1/Bodies/Body  RConnTagsString=CS2  UpdateFromCAD=on  PMImportedID=pin50mm-5  DialogClass=MechanicalBodyBlock  Mass=0.00250309  MassUnits=kg  InertiaUnits=kg*m^2  Inertia=[5.27329e-07,0,0;0,5.27329e-07,0;0,0,1.99599e-08]  Shape=Cylinder  ShapeDims=[1 1]  ShapeUnits=m  ShapeUse=false  Density=1  DensityUnits=kg/m^3  DensityUse=false  GraphicsMode=GFXFILE  GraphicsFileName=GripperForSimulink - pin50mm-5.STL  BodyColorSelMode=COLORPALETTE  BodyColor=[0.666667;0.698039;0.768627]  AttachedToCS=CS1  CG=Right$CG$[0.0560713 0.043243 0.0235926]$WORLD$WORLD$m$[1 0 0;0 1 0;0 0 1]$3x3 Transform$rad$WORLD$false$pin50mm-5::CG(AUTOGEN)  WorkingFrames=Right$CS1$[0.0560713 0.043243 -0.00140736]$WORLD$WORLD$m$[1 0 0;0 1 0;0 0 1]$3x3 Transform$rad$WORLD$false$pin50mm-5::CS1(AUTOGEN)#Right$CS2$[0.0560713 0.043243 0.0485926]$WORLD$WORLD$m$[1 0 0;0 1 0;0 0 1]$3x3 Transform$rad$WORLD$true$link2-3:-:pin50mm-5::pin50mm-5(AUTOGEN)  CGPos=[0.0560713 0.043243 0.0235926]  CGRot=[1 0 0;0 1 0;0 0 1]  CS0Pos=[]  CS0Rot=[]  CS1Pos=[0.0560713 0.043243 -0.00140736]  CS1Rot=[1 0 0;0 1 0;0 0 1]  CS2Pos=[0.0560713 0.043243 0.0485926]  CS2Rot=[1 0 0;0 1 0;0 0 1]  CS3Pos=[]  CS3Rot=[]  CS4Pos=[]  CS4Rot=[]  CS5Pos=[]  CS5Rot=[]  CS6Pos=[]  CS6Rot=[]  CS7Pos=[]  CS7Rot=[]  CS8Pos=[]  CS8Rot=[]  CS9Pos=[]  CS9Rot=[]  CS10Pos=[]  CS10Rot=[]  CS11Pos=[]  CS11Rot=[]  CS12Pos=[]  CS12Rot=[]  CS13Pos=[]  CS13Rot=[]  CS14Pos=[]  CS14Rot=[]  CS15Pos=[]  CS15Rot=[]  CS16Pos=[]  CS16Rot=[]  CS17Pos=[]  CS17Rot=[]  CS18Pos=[]  CS18Rot=[]  CS19Pos=[]  CS19Rot=[]  CS20Pos=[]  CS20Rot=[]
  pin50mm-6 : mblibv1/Bodies/Body  LConnTagsString=CS2  UpdateFromCAD=on  PMImportedID=pin50mm-6  DialogClass=MechanicalBodyBlock  Mass=0.00250309  MassUnits=kg  InertiaUnits=kg*m^2  Inertia=[5.27329e-07,0,0;0,5.27329e-07,0;0,0,1.99599e-08]  Shape=Cylinder  ShapeDims=[1 1]  ShapeUnits=m  ShapeUse=false  Density=1  DensityUnits=kg/m^3  DensityUse=false  GraphicsMode=GFXFILE  GraphicsFileName=GripperForSimulink - pin50mm-6.STL  BodyColorSelMode=COLORPALETTE  BodyColor=[0.666667;0.698039;0.768627]  AttachedToCS=CS1  CG=Right$CG$[0.0480334 0.0678885 0.0233426]$WORLD$WORLD$m$[1 0 0;0 1 0;0 0 1]$3x3 Transform$rad$WORLD$false$pin50mm-6::CG(AUTOGEN)  WorkingFrames=Right$CS1$[0.0480334 0.0678885 -0.00165736]$WORLD$WORLD$m$[1 0 0;0 1 0;0 0 1]$3x3 Transform$rad$WORLD$false$pin50mm-6::CS1(AUTOGEN)#Left$CS2$[0.0480334 0.0678885 -0.00165736]$WORLD$WORLD$m$[1 0 0;0 1 0;0 0 1]$3x3 Transform$rad$WORLD$true$link3-1:-:pin50mm-6::pin50mm-6(AUTOGEN)  CGPos=[0.0480334 0.0678885 0.0233426]  CGRot=[1 0 0;0 1 0;0 0 1]  CS0Pos=[]  CS0Rot=[]  CS1Pos=[0.0480334 0.0678885 -0.00165736]  CS1Rot=[1 0 0;0 1 0;0 0 1]  CS2Pos=[0.0480334 0.0678885 -0.00165736]  CS2Rot=[1 0 0;0 1 0;0 0 1]  CS3Pos=[]  CS3Rot=[]  CS4Pos=[]  CS4Rot=[]  CS5Pos=[]  CS5Rot=[]  CS6Pos=[]  CS6Rot=[]  CS7Pos=[]  CS7Rot=[]  CS8Pos=[]  CS8Rot=[]  CS9Pos=[]  CS9Rot=[]  CS10Pos=[]  CS10Rot=[]  CS11Pos=[]  CS11Rot=[]  CS12Pos=[]  CS12Rot=[]  CS13Pos=[]  CS13Rot=[]  CS14Pos=[]  CS14Rot=[]  CS15Pos=[]  CS15Rot=[]  CS16Pos=[]  CS16Rot=[]  CS17Pos=[]  CS17Rot=[]  CS18Pos=[]  CS18Rot=[]  CS19Pos=[]  CS19Rot=[]  CS20Pos=[]  CS20Rot=[]
  Displacement : PMIOPort  Port=1  Side=Left
  position : Outport
  velocity : Outport  Port=2
  acceleration : Outport  Port=3
  wires:
  Joint Sensor/1 -> position/1
  Joint Sensor/2 -> velocity/1
  Joint Sensor/3 -> acceleration/1
  connections:
  Revolute11/LConn1 -- base-1/RConn5
  Revolute11/RConn1 -- pin1-5/LConn1
  link2-1/LConn1 -- Revolute3/RConn1
  base-1/RConn7 -- Cylindrical6/LConn1
  RootPart/RConn2 -- Weld1/LConn1
  Revolute6/LConn1 -- base-1/RConn2
  pin1-2/LConn1 -- Revolute5/RConn1
  link2-3/LConn1 -- Revolute7/RConn1
  Cylindrical1/LConn1 -- base-1/RConn6
  Revolute3/LConn1 -- base-1/RConn3
  Revolute5/LConn1 -- base-1/RConn1
  RootPart/RConn1 -- Weld/LConn1
  Revolute7/LConn1 -- base-1/RConn4
  driveshaft-2/LConn1 -- Cylindrical1/RConn1
  Weld/RConn1 -- Part8^GripperForSimulink-1/LConn1
  Weld1/RConn1 -- base-1/LConn1
  link3-1/LConn1 -- Revolute6/RConn1
  Cylindrical6/RConn1 -- link4-1/LConn1
  Revolute17/LConn1 -- base-1/RConn8
  link3-2/LConn1 -- Revolute17/RConn1
  Revolute16/RConn1 -- link2-2/LConn1
  Revolute16/LConn1 -- base-1/RConn9
  Revolute25/LConn1 -- pin50mm-3/RConn1
  Revolute9/LConn1 -- link3-1/RConn2
  Revolute13/LConn1 -- link1-1/RConn1
  Revolute8/LConn1 -- link3-1/RConn1
  Revolute26/LConn1 -- link2-2/RConn1
  Revolute13/RConn1 -- link3-1/LConn2
  Revolute8/RConn1 -- pin50mm-6/LConn1
  Revolute25/RConn1 -- link2-4/LConn1
  Revolute26/RConn1 -- pin50mm-3/LConn1
  Revolute9/RConn1 -- pin15mm-2/LConn1
  Revolute23/LConn1 -- link2-2/RConn2
  grip-1/RConn1 -- Revolute10/LConn1
  Revolute28/LConn1 -- link1-1/RConn2
  Revolute28/RConn1 -- link4-1/LConn2
  Revolute20/LConn1 -- link3-2/RConn1
  grip-1/RConn2 -- Revolute4/LConn1
  grip-2/LConn1 -- Revolute20/RConn1
  link2-1/LConn2 -- Revolute4/RConn1
  link3-1/LConn3 -- Revolute10/RConn1
  Revolute18/RConn1 -- link1-2/LConn1
  Revolute19/LConn1 -- link1-2/RConn1
  link4-1/RConn3 -- Planar/LConn1
  Revolute24/LConn1 -- pin50mm-1/RConn1
  Revolute21/RConn1 -- pin15mm-4/LConn1
  Revolute21/LConn1 -- link3-2/RConn2
  Revolute22/RConn1 -- pin50mm-2/LConn1
  Revolute/RConn1 -- link2-3/LConn2
  Revolute27/RConn1 -- pin50mm-1/LConn1
  Revolute22/LConn1 -- link3-2/RConn3
  link3-2/LConn2 -- Revolute19/RConn1
  Revolute23/RConn1 -- grip-2/LConn2
  Revolute14/RConn1 -- pin15mm-1/LConn1
  Planar/RConn1 -- driveshaft-2/LConn2
  Revolute15/RConn1 -- pin15mm-3/LConn1
  Revolute27/LConn1 -- link2-2/RConn3
  Revolute1/RConn1 -- link2-3/LConn3
  Revolute/LConn1 -- pin50mm-4/RConn1
  Revolute2/RConn1 -- link2-3/LConn4
  Revolute15/LConn1 -- link4-1/RConn2
  Revolute1/LConn1 -- pin50mm-5/RConn1
  Revolute14/LConn1 -- link4-1/RConn1
  Revolute24/RConn1 -- link2-4/LConn2
  Revolute2/LConn1 -- grip-1/RConn3
  Revolute18/LConn1 -- link4-1/RConn4
  RootGround/RConn1 -- Weld2/LConn1
  Weld2/RConn1 -- RootPart/LConn1
  RootGround/LConn1 -- Machine Environment/RConn1
  Joint Sensor/LConn1 -- Cylindrical1/RConn2
  Displacement/RConn1 -- Cylindrical1/LConn2
